simulink model "ACT_ur10"  (R2021b)
(part 6 of 6)

t5571 = -t4d.*(t4257+t4274-t5096+t14.*(t1862+t2375+t330.*(-t496-t547+t615+t623+t755+t8.*t37.*(t100-t364))+t2124.*(t100-t364)));
t5573 = t5572.*t2d;
t5574 = t5572.*t3d;
t5575 = t5572.*t4d;
t5584 = t5583.*t2d;
t5585 = t5583.*t3d;
t5586 = t5583.*t4d;
t5604 = t5601.*t6d;
t5612 = t2665+t2848+t2884+t2931+t3229+t3273+t4524+t4593+t4609;
t5616 = t2188+t2614+t2617+t2986+t3283+t3295+t4605+t4731+t4734;
t5624 = t3661+t3691+t5369+t5376;
t5630 = t3424+t3700+t3759+t5296+t5297;
t5633 = t4477+t4478+t5280+t5288;
t5637 = t2691+t2900+t2902+t4527+t4657+t4660+t5218;
t5641 = t4203+t4230+t4424+t4792+t4813+t4880;
t5642 = t2721+t2899+t2971+t4564+t4684+t4689+t5218;
t5648 = t2814+t3138+t3144+t3608+t3818+t3820+t5101+t5117;
t5652 = t2661+t2842+t2867+t4519+t4614+t4623+t4635+t4649;
t5653 = t2815+t3139+t3143+t3653+t3865+t3914+t5126+t5139;
t5654 = t2970+t3100+t3125+t4209+t4248+t4746+t4795+t4807;
t5662 = t2994+t3076+t3165+t4209+t4248+t4758+t4816+t4839;
t5663 = t2709+t2882+t2901+t4542+t4610+t4619+t4673+t4679;
t5664 = t2887+t3181+t3187+t3673+t3969+t4021+t5135+t5162;
t5665 = -t2d.*(t2845+t3136-t3187-t3673-t3969+t4015-t5135+t5158./2.0);
t5666 = -t3d.*(t2845+t3136-t3187-t3673-t3969+t4015-t5135+t5158./2.0);
t5667 = -t4d.*(t2845+t3136-t3187-t3673-t3969+t4015-t5135+t5158./2.0);
t5669 = t5668.*t1d;
t5671 = t833+t4661+t4662+t4663+t5152+t5231;
t5672 = -t5d.*(t3413+t3663-t3717-t4462-t4463+t4501+t4633./2.0+t4655./2.0);
t5678 = t3009+t3124+t3162+t4406+t4419+t4766+t4852+t4857;
t5681 = t2054+t2427+t2463+t2963+t2982+t3140+t3166+t3337+t3373+t4750+t4817+t4829;
t5688 = t2205+t5240+t5241+t5242+t5272;
t5689 = t2205+t5237+t5238+t5239+t5272;
t5690 = t3670+t3839+t3858+t3960+t3967+t5048+t5132+t5154;
t5693 = -t6d.*(-t2810-t3112+t3146+t3629+t3961-t5142+(t330.*(t1862+t2375+t330.*(-t496-t547+t615+t623+t755+t8.*t37.*(t100-t364))+t2124.*(t100-t364)))./2.0+(t18.*t39.*(t1873+t2355+t2471+t3579))./2.0+(t38.*t39.*(t2068-t2488))./2.0);
t5694 = t6d.*(-t2810-t3112+t3146+t3629+t3961-t5142+(t330.*(t1862+t2375+t330.*(-t496-t547+t615+t623+t755+t8.*t37.*(t100-t364))+t2124.*(t100-t364)))./2.0+(t18.*t39.*(t1873+t2355+t2471+t3579))./2.0+(t38.*t39.*(t2068-t2488))./2.0);
t5695 = t3694+t3926+t3955+t3958+t4006+t5062+t5167+t5183;
t5697 = t3672+t3928+t3975+t4961+t5074+t5186+t5190;
t5700 = -t6d.*(t3735+t3991+t4006./2.0-t4996+t5062./2.0+t5181+t5194);
t5701 = t6d.*(t3735+t3991+t4006./2.0-t4996+t5062./2.0+t5181+t5194);
t5702 = t2850+t3279+t3314+t3736+t3996+t4013+t5082+t5195+t5201;
t5707 = t3552+t3863+t3915+t4729+t4742+t5038+t5105+t5119;
t5708 = t1357+t4987+t4988+t4989+t5338+t5375;
t5712 = t3597+t3900+t3947+t4037+t4278+t4310+t5041+t5110+t5131;
t5713 = t3379+t3632+t3703+t4490+t4633+t4655+t5284+t5294;
t5724 = -t2d.*(t3408-t3662+t3702-t4498+t4675-t5371+t5378+t255.*(t1929-t1996+t2033+t1187.*(t101-t401)));
t5725 = -t3d.*(t3408-t3662+t3702-t4498+t4675-t5371+t5378+t255.*(t1929-t1996+t2033+t1187.*(t101-t401)));
t5726 = -t4d.*(t3408-t3662+t3702-t4498+t4675-t5371+t5378+t255.*(t1929-t1996+t2033+t1187.*(t101-t401)));
t5728 = t3659+t3913+t3917+t5051+t5073+t5086+t5176+t5182;
t5731 = t3420+t5316+t5317+t5318+t5473;
t5732 = -t5d.*(t3398+t5470+t2d.*(t1046+t1185+t1189+t1434-t3519+t158.*t789+t515.*t789+(t8.*(t1609-t2416))./2.0)+t3d.*(t1046+t1185+t1189+t1434-t3519+t158.*t789+t515.*t789+(t8.*(t1609-t2416))./2.0)+t4d.*(t1046+t1185+t1189+t1434-t3519+t158.*t789+t515.*t789+(t8.*(t1609-t2416))./2.0));
t5733 = t5d.*(t3398+t5470+t2d.*(t1046+t1185+t1189+t1434-t3519+t158.*t789+t515.*t789+(t8.*(t1609-t2416))./2.0)+t3d.*(t1046+t1185+t1189+t1434-t3519+t158.*t789+t515.*t789+(t8.*(t1609-t2416))./2.0)+t4d.*(t1046+t1185+t1189+t1434-t3519+t158.*t789+t515.*t789+(t8.*(t1609-t2416))./2.0));
t5741 = -t5d.*(-t2846-t3274-t3277-t3710+t3971+t4036+t4343+t4369+t5156+(t37.*(-t1537+t1983+t3892+t18.*t37.*(t544-t1021+t330.*(t100-t364))))./2.0+(t8.*t37.*(t1070.*(t100-t364)+t330.*(t544-t1021+t330.*(t100-t364))))./2.0+(t14.*t39.*(t1585+t2193-t4001+t38.*t39.*(t544-t1021+t330.*(t100-t364))))./2.0);
t5742 = t5d.*(-t2846-t3274-t3277-t3710+t3971+t4036+t4343+t4369+t5156+(t37.*(-t1537+t1983+t3892+t18.*t37.*(t544-t1021+t330.*(t100-t364))))./2.0+(t8.*t37.*(t1070.*(t100-t364)+t330.*(t544-t1021+t330.*(t100-t364))))./2.0+(t14.*t39.*(t1585+t2193-t4001+t38.*t39.*(t544-t1021+t330.*(t100-t364))))./2.0);
t5765 = t4210+t4240+t4364+t4413+t4446+t5356+t5377+t5382;
t5766 = t4116+t4247+t4291+t4311+t4484+t4489+t5264+t5293+t5299;
t5768 = t4373+t4417+t4429+t4441+t4445+t5355+t5384+t5388;
t2922 = -t2903;
t2924 = -t2905;
t3470 = -t3447;
t4821 = t4808.*t5d;
t4823 = t4809.*t5d;
t4910 = t4904.*t2d;
t4911 = t4904.*t3d;
t4912 = t4904.*t4d;
t4965 = -t4963;
t4999 = t2888+t3255+t3300;
t5205 = t1247+t1648+t1649+t2301+t2689+t2707;
t5232 = t3436+t3772+t3795;
t5274 = t5273.*t5d;
t5332 = t5326.*t2d;
t5333 = t5326.*t3d;
t5334 = t5326.*t4d;
t5339 = t5331.*t2d;
t5340 = t5331.*t3d;
t5341 = t5331.*t4d;
t5347 = -t5344;
t5390 = t5387.*t2d;
t5391 = t5387.*t3d;
t5392 = t5387.*t4d;
t5405 = t5404.*t5d;
t5412 = t5411.*t1d;
t5415 = t2907+t3303+t3333+t4915;
t5417 = -t6d.*(-t2907+t3293+t3324-t3867+t14.*(t1070.*(t100-t364)+t330.*(t544-t1021+t330.*(t100-t364))));
t5420 = t5416.*t5d;
t5421 = t6d.*(-t2907+t3293+t3324-t3867+t14.*(t1070.*(t100-t364)+t330.*(t544-t1021+t330.*(t100-t364))));
t5423 = t5419.*t5d;
t5444 = t5443.*t2d;
t5445 = t5443.*t3d;
t5446 = t5443.*t4d;
t5456 = t301+t4031+t4032+t4033+t4791;
t5472 = -t5469;
t5474 = -t5471;
t5479 = t5477.*t5d;
t5488 = t5487.*t2d;
t5489 = t5487.*t3d;
t5490 = t5487.*t4d;
t5493 = t5492.*t5d;
t5495 = t3448+t3814+t3837+t5243;
t5496 = -t6d.*(-t3448+t3801+t3824-t4411+t14.*(t2578.*(t100-t364)+t609.*(t544-t1021+t330.*(t100-t364))));
t5497 = t6d.*(-t3448+t3801+t3824-t4411+t14.*(t2578.*(t100-t364)+t609.*(t544-t1021+t330.*(t100-t364))));
t5499 = t5498.*t6d;
t5509 = t3438+t3664+t3731+t4594+t4608;
t5510 = t5508.*t5d;
t5518 = t2468+t2668+t2683+t2946+t4184+t4320+t4323;
t5519 = t2466+t2669+t2676+t2947+t4181+t4316+t4318;
t5524 = t2099+t2476+t2506+t3001+t3353+t3396+t5147;
t5527 = t5525.*t6d;
t5530 = t5529.*t2d;
t5531 = t5529.*t3d;
t5532 = t5529.*t4d;
t5535 = t5533.*t2d;
t5536 = t5533.*t3d;
t5537 = t5533.*t4d;
t5538 = t5534.*t2d;
t5539 = t5534.*t3d;
t5540 = t5534.*t4d;
t5541 = t4405+t5455;
t5547 = t2923+t3217+t3239+t3713+t3998+t4035+t4422;
t5553 = t5550.*t5d;
t5563 = t4044+t4305+t4329+t4717+t4725;
t5566 = t5565.*t5d;
t5568 = t4263+t4289+t5096+t5104;
t5587 = t2872+t3190+t3201+t3646+t3842+t3847+t4245+t4262;
t5590 = t2873+t3184+t3205+t3689+t3891+t3946+t4235+t4249;
t5592 = t2079+t2243+t2363+t3294+t3549+t3576+t4814+t4835;
t5599 = t4124+t4344+t4350+t4363+t4421+t4433;
t5606 = t4340+t4496+t4497+t4918+t4919;
t5609 = t2625+t2808+t2830+t3952+t3977+t4515+t4586+t4601;
t5613 = t5612.*t5d;
t5615 = t3990+t4071+t4084+t4694+t4716+t4986;
t5631 = t5630.*t5d;
t5634 = t5633.*t2d;
t5635 = t5633.*t3d;
t5636 = t5633.*t4d;
t5639 = t3446+t3645+t3655+t3714+t3742+t4507+t4686+t4699;
t5643 = t5642.*t6d;
t5649 = t5648.*t2d;
t5650 = t5648.*t3d;
t5651 = t5648.*t4d;
t5655 = t5653.*t2d;
t5656 = t5653.*t3d;
t5657 = t5653.*t4d;
t5658 = t2886+t3180+t3188+t3631+t3911+t3964+t5127+t5134;
t5670 = t3425+t3676+t3717+t4462+t4463+t4502+t4640+t4659;
t5673 = t5671.*t1d;
t5677 = t3017+t3137+t3240+t3411+t3793+t3816+t4772+t4854+t4866;
t5682 = t5681.*t5d;
t5683 = t2080+t2428+t2520+t2968+t3004+t3126+t3192+t3338+t3339+t4767+t4834+t4847;
t5692 = t3644+t3932+t3973+t4962+t5043+t5142+t5171;
t5698 = t5697.*t6d;
t5699 = t3748+t4000+t4012+t4996+t5066+t5185+t5199;
t5703 = t5702.*t6d;
t5704 = t1356+t4972+t4973+t4974+t5329+t5367;
t5709 = t5708.*t1d;
t5715 = t5713.*t2d;
t5716 = t5713.*t3d;
t5717 = t5713.*t4d;
t5723 = t3434+t3662+t3723+t4498+t4677+t4681+t5371+t5380;
t5727 = t3616+t3886+t3945+t5040+t5080+t5089+t5130+t5163;
t5730 = -t5d.*(-t3389+t5469+t2d.*(t1045+t1183+t1184+t1440-t3514+t155.*t788+t508.*t788+(t14.*(t1597-t2409))./2.0)+t3d.*(t1045+t1183+t1184+t1440-t3514+t155.*t788+t508.*t788+(t14.*(t1597-t2409))./2.0)+t4d.*(t1045+t1183+t1184+t1440-t3514+t155.*t788+t508.*t788+(t14.*(t1597-t2409))./2.0));
t5734 = t3386+t3665+t3719+t4123+t4276+t4313+t5266+t5310+t5322;
t5740 = t2846+t3274+t3277+t3710+t3985+t3997+t4043+t4354+t4380+t5057+t5148+t5160;
t5743 = t2847+t3276+t3316+t3711+t3988+t3992+t4053+t4358+t4359+t5075+t5161+t5174;
t5747 = -t2d.*(t3241+t5471+t2d.*(t3350-t3369)+t3d.*(t3350-t3369)+t4d.*(t3350-t3369)+t6d.*(t2098+t2330./2.0+t2351+t3264./2.0-t3507+t3541-t4797));
t5748 = -t3d.*(t3241+t5471+t2d.*(t3350-t3369)+t3d.*(t3350-t3369)+t4d.*(t3350-t3369)+t6d.*(t2098+t2330./2.0+t2351+t3264./2.0-t3507+t3541-t4797));
t5749 = -t4d.*(t3241+t5471+t2d.*(t3350-t3369)+t3d.*(t3350-t3369)+t4d.*(t3350-t3369)+t6d.*(t2098+t2330./2.0+t2351+t3264./2.0-t3507+t3541-t4797));
t5750 = t2d.*(t3241+t5471+t2d.*(t3350-t3369)+t3d.*(t3350-t3369)+t4d.*(t3350-t3369)+t6d.*(t2098+t2330./2.0+t2351+t3264./2.0-t3507+t3541-t4797));
t5751 = t3d.*(t3241+t5471+t2d.*(t3350-t3369)+t3d.*(t3350-t3369)+t4d.*(t3350-t3369)+t6d.*(t2098+t2330./2.0+t2351+t3264./2.0-t3507+t3541-t4797));
t5752 = t4d.*(t3241+t5471+t2d.*(t3350-t3369)+t3d.*(t3350-t3369)+t4d.*(t3350-t3369)+t6d.*(t2098+t2330./2.0+t2351+t3264./2.0-t3507+t3541-t4797));
t5758 = t4106+t4223+t4260+t4927+t4928+t5261+t5287+t5295;
t5767 = t5766.*t5d;
t5769 = t3437+t3823+t3825+t4384+t4444+t4465+t5359+t5386+t5393;
t5771 = t1792+t5300+t5301+t5302+t5431+t5448;
t5774 = t5399+t5731;
t5775 = -t5d.*(t3398-t5399+t5470+t2d.*(t1046+t1185+t1189+t1434-t3519+t158.*t789+t515.*t789+(t8.*(t1609-t2416))./2.0)+t3d.*(t1046+t1185+t1189+t1434-t3519+t158.*t789+t515.*t789+(t8.*(t1609-t2416))./2.0)+t4d.*(t1046+t1185+t1189+t1434-t3519+t158.*t789+t515.*t789+(t8.*(t1609-t2416))./2.0));
t5776 = t5d.*(t3398-t5399+t5470+t2d.*(t1046+t1185+t1189+t1434-t3519+t158.*t789+t515.*t789+(t8.*(t1609-t2416))./2.0)+t3d.*(t1046+t1185+t1189+t1434-t3519+t158.*t789+t515.*t789+(t8.*(t1609-t2416))./2.0)+t4d.*(t1046+t1185+t1189+t1434-t3519+t158.*t789+t515.*t789+(t8.*(t1609-t2416))./2.0));
t5785 = t3435+t3773+t3836+t4328+t4382+t4430+t4455+t4511+t4516+t5357+t5379+t5383;
t5003 = t4999.*t6dd;
t5208 = t5205.*t6d;
t5233 = t5232.*t6dd;
t5275 = -t5274;
t5394 = -t5390;
t5395 = -t5391;
t5396 = -t5392;
t5407 = -t5405;
t5414 = -t5412;
t5424 = -t5420;
t5425 = -t5423;
t5457 = t5456.*t1d;
t5500 = -t5499;
t5512 = -t5510;
t5520 = t5518.*t5d;
t5521 = t5519.*t5d;
t5526 = t5524.*t6d;
t5544 = t2922+t3223+t3233+t3660+t3957+t3995+t4423;
t5548 = t5547.*t6d;
t5554 = -t5553;
t5564 = t5563.*t5d;
t5567 = -t5566;
t5588 = t5587.*t5d;
t5591 = t5590.*t5d;
t5594 = t5592.*t2d;
t5595 = t5592.*t3d;
t5596 = t5592.*t4d;
t5598 = t2924+t3315+t3317+t4051+t4365+t4383+t4895;
t5602 = t5599.*t6d;
t5607 = t5606.*t5d;
t5614 = -t5613;
t5632 = -t5631;
t5640 = t5639.*t6d;
t5644 = t3470+t3794+t3855+t4191+t4214+t4347+t4518+t4523;
t5646 = t1083+t4821+t5191+t5192+t5193;
t5647 = t1084+t4823+t5196+t5197+t5198;
t5659 = t5658.*t2d;
t5660 = t5658.*t3d;
t5661 = t5658.*t4d;
t5674 = t3010+t3182+t3204+t4756+t4849+t4851+t5232;
t5679 = t5677.*t6d;
t5684 = t5683.*t5d;
t5705 = t5704.*t1d;
t5710 = -t5709;
t5729 = t3389+t5319+t5320+t5321+t5472;
t5735 = t5734.*t6d;
t5736 = t2874+t5007+t5008+t5009+t5277+t5493;
t5744 = t5743.*t5d;
t5746 = t3257+t4637+t4638+t4639+t5474+t5504;
t5753 = t3296+t4690+t4691+t4692+t5479+t5507;
t5755 = -t2d.*(t3270-t5479-t5507+t2d.*(t3442+(t14.*(t1864-t2028))./2.0)+t3d.*(t3442+(t14.*(t1864-t2028))./2.0)+t4d.*(t3442+(t14.*(t1864-t2028))./2.0));
t5756 = -t3d.*(t3270-t5479-t5507+t2d.*(t3442+(t14.*(t1864-t2028))./2.0)+t3d.*(t3442+(t14.*(t1864-t2028))./2.0)+t4d.*(t3442+(t14.*(t1864-t2028))./2.0));
t5757 = -t4d.*(t3270-t5479-t5507+t2d.*(t3442+(t14.*(t1864-t2028))./2.0)+t3d.*(t3442+(t14.*(t1864-t2028))./2.0)+t4d.*(t3442+(t14.*(t1864-t2028))./2.0));
t5770 = t5769.*t6d;
t5772 = t5771.*t1d;
t5786 = t5785.*t5d;
t5792 = t3393+t5484+t5485+t5486+t5497+t5511;
t5794 = t4630+t5535+t5536+t5537+t5618;
t5797 = t1031+t2500+t2502+t2504+t3378+t5246+t5247+t5248+t5349+t5730;
t5798 = t1081+t2499+t2501+t2503+t3358+t5252+t5253+t5254+t5347+t5733;
t5799 = t2890+t5422+t5530+t5531+t5532+t5552;
t5811 = -t5d.*(t4520+t5613+t2d.*(-t2021+t2249+t3374+t3395+t4569-t4577+t37.*(t1580+t2001)+t8.*t37.*t1503.*(t100-t364))+t3d.*(-t2021+t2249+t3374+t3395+t4569-t4577+t37.*(t1580+t2001)+t8.*t37.*t1503.*(t100-t364))+t4d.*(-t2021+t2249+t3374+t3395+t4569-t4577+t37.*(t1580+t2001)+t8.*t37.*t1503.*(t100-t364))+t6d.*(t2675+t2885-t3385+t3633-t3680-t4527+t4656-t4657+(t892.*t2198)./2.0));
t5812 = t4543+t5560+t5561+t5562+t5622+t5643;
t5823 = t5044+t5649+t5650+t5651+t5694+t5718;
t5825 = t5070+t5655+t5656+t5657+t5698+t5721;
t5236 = -t5233;
t5522 = -t5520;
t5528 = -t5526;
t5545 = t5544.*t6d;
t5549 = -t5548;
t5576 = t2203+t3775+t3776+t3777+t5407;
t5589 = -t5588;
t5593 = -t5591;
t5600 = t5598.*t6d;
t5605 = -t5602;
t5608 = -t5607;
t5645 = t5644.*t6d;
t5676 = t5674.*t6d;
t5680 = -t5679;
t5706 = -t5705;
t5722 = t5208+t5689;
t5737 = -t5735;
t5738 = t5736.*t6d;
t5745 = -t5744;
t5754 = t2129+t5275+t5440+t5441+t5442;
t5759 = t4219+t5332+t5333+t5334+t5521;
t5791 = t2984+t5425+t5450+t5451+t5452+t5527;
t5793 = t3393+t5488+t5489+t5490+t5497+t5512;
t5795 = t5794.*t5d;
t5800 = t2834+t5421+t5538+t5539+t5540+t5554;
t5801 = t4510+t5335+t5336+t5337+t5640+t5672;
t5809 = t4079+t5567+t5573+t5574+t5575+t5604;
t5810 = t4525+t5556+t5557+t5558+t5614+t5638;
t5813 = t5812.*t5d;
t5815 = t3327+t5500+t5625+t5626+t5627+t5632;
t5824 = t5823.*t5d;
t5826 = t5825.*t5d;
t5827 = t5071+t5659+t5660+t5661+t5701+t5742;
t5830 = -t6d.*(t5088-t5703+t5744+t2d.*(t2845+t3136-t3187-t3673-t3969+t4015-t5135+t5158./2.0)+t3d.*(t2845+t3136-t3187-t3673-t3969+t4015-t5135+t5158./2.0)+t4d.*(t2845+t3136-t3187-t3673-t3969+t4015-t5135+t5158./2.0));
t5835 = t5363+t5724+t5725+t5726+t5770+t5786;
t5546 = -t5545;
t5577 = t5576.*t2d;
t5578 = t5576.*t3d;
t5579 = t5576.*t4d;
t5603 = -t5600;
t5739 = -t5738;
t5760 = t4211+t5339+t5340+t5341+t5522;
t5761 = t5759.*t5d;
t5781 = t3692+t4910+t4911+t4912+t5549+t5593;
t5790 = t2939+t5424+t5444+t5445+t5446+t5528;
t5796 = -t5795;
t5802 = t5801.*t2d;
t5803 = t5801.*t3d;
t5804 = t5801.*t4d;
t5814 = -t5813;
t5816 = t4753+t5584+t5585+t5586+t5676+t5682;
t5819 = t4761+t5594+t5595+t5596+t5680+t5684;
t5821 = t4368+t5608+t5634+t5635+t5636+t5645;
t5828 = t5827.*t6d;
t5829 = t5095+t5665+t5666+t5667+t5703+t5745;
t5832 = t5271+t5715+t5716+t5717+t5737+t5767;
t5836 = t5835.*t6d;
t5580 = -t5577;
t5581 = -t5578;
t5582 = -t5579;
t5762 = t5760.*t5d;
t5763 = -t5761;
t5777 = t3657+t4884+t4885+t4886+t5546+t5589;
t5782 = t5781.*t2d;
t5783 = t5781.*t3d;
t5784 = t5781.*t4d;
t5805 = -t5802;
t5806 = -t5803;
t5807 = -t5804;
t5808 = t4062+t5564+t5569+t5570+t5571+t5603;
t5817 = t5816.*t6d;
t5820 = t5819.*t6d;
t5822 = t1081+t2499+t2501+t2503+t3236+t3358+t5394+t5395+t5396+t5414+t5739+t5776;
t5833 = t5832.*t5d;
t5837 = -t5836;
t5764 = -t5762;
t5778 = t5777.*t2d;
t5779 = t5777.*t3d;
t5780 = t5777.*t4d;
t5788 = t982+t2997+t3725+t3727+t3729+t5324+t5763;
t5818 = -t5817;
t5831 = t2130+t4009+t4010+t4011+t4557+t5457+t5580+t5581+t5582+t5796;
t5834 = -t5833;
t5839 = t2026+t3635+t3637+t3639+t4399+t4479+t5673+t5755+t5756+t5757+t5814+t5820;
t5841 = t2759+t4447+t4448+t4449+t4966+t5004+t5710+t5782+t5783+t5784+t5826+t5830;
t5789 = t983+t2998+t3726+t3728+t3730+t5323+t5764;
t5838 = t1940+t3636+t3638+t3640+t4400+t4480+t5669+t5750+t5751+t5752+t5811+t5818;
t5840 = t2758+t4434+t4436+t4438+t4965+t5003+t5706+t5778+t5779+t5780+t5824+t5828;
t5842 = t3361+t4818+t4819+t4820+t5220+t5236+t5772+t5805+t5806+t5807+t5834+t5837;
et1 = -t2d.*(t4d.*(t2467+t2490+t3177+t3185)-t3d.*(t2956+t2989+t3349+t3351)-t2d.*(-t8.*t1302.*t2174+t14.*t1302.*t2168+t8.*t1321.*t2659+t14.*t1321.*t2655)+t5d.*(t2070+t2085-t2937-t2951))+t1d.*(-t5d.*(t706.*t2655.*2.0+t723.*t2659.*2.0)+t4d.*(t1288.*t2655.*2.0-t1298.*t2659.*2.0)+t3d.*(t1962.*t2655.*2.0-t1977.*t2659.*2.0)+t2d.*(t2168.*t2655.*2.0-t2174.*t2659.*2.0))+t4491.*t4dd+t4596.*t3dd+t4695.*t2dd-t5018.*t5dd-t4d.*(t3d.*(t2606+t2642+t3177+t3185)+t2d.*(t2745+t2775+t3177+t3185)+t4d.*(t3177+t3185-t14.*t687.*t1288+t8.*t687.*t1298)+t5d.*(t1547+t1574-t2937-t2951));
et2 = -t3d.*(t4d.*(t2286+t2346+t3177+t3185)-t2d.*(t2995+t3007+t3349+t3351)-t3d.*(t3349+t3351+t14.*t1036.*t1962-t8.*t1036.*t1977)+t5d.*(t1837+t1866-t2937-t2951))+t1dd.*(t2655.^2+t2659.^2)+t5d.*(t2d.*(t3840+t3875+t4579+t4591)+t4d.*(t3331+t4579+t4591+t1288.*(t859-t1704))+t3d.*(t3712+t4579+t4591+t1962.*(t859-t1704))+t5d.*(t723.*t2507+t1399.*t2655-t706.*(t859-t1704)-t2659.*(t441-t846)));
et3 = -t2d.*(t4d.*(t3183+t3214+t3781+t3785)+t3d.*(t3557+t3574+t3972+t3976)-t2d.*(-t8.*t2173.*t2279+t14.*t2167.*t2279+t8.*t2357.*t2658+t14.*t2357.*t2654)+t5d.*(t2862+t2876-t3359-t3360))-t6dd.*(t2658.*(t873-t2434)+t2654.*(t910-t2473))+t1d.*(-t5d.*(t705.*t2654.*2.0+t721.*t2658.*2.0)+t4d.*(t1287.*t2654.*2.0-t1297.*t2658.*2.0)+t3d.*(t1961.*t2654.*2.0-t1976.*t2658.*2.0)+t2d.*(t2167.*t2654.*2.0-t2173.*t2658.*2.0))+t4878.*t4dd+t4946.*t3dd+t4967.*t2dd-t5219.*t5dd-t5787.*t6d+t5d.*(t2d.*(t4166+t4189+t4931+t4938)+t5d.*(t721.*t3230+t705.*t3251+t2123.*t2654+t2169.*t2658)+t4d.*(t3923-t3936+t4931+t4938)+t3d.*(t4125-t4128+t4931+t4938));
et4 = -t4d.*(t3d.*(t3308+t3321+t3781+t3785)+t2d.*(t3415+t3445+t3781+t3785)+t4d.*(t3781+t3785-t14.*t1287.*t1807+t8.*t1297.*t1807)+t5d.*(t2509+t2527-t3359-t3360))-t3d.*(t4d.*(t3035+t3069+t3781+t3785)+t2d.*(t3575+t3617+t3972+t3976)+t3d.*(t3972+t3976-t14.*t1961.*t2113+t8.*t1976.*t2113)+t5d.*(t2708+t2718-t3359-t3360))+t1dd.*(t2654.^2+t2658.^2);
et5 = -t5dd.*(t37.*t418+t14.*t496.*t641+t8.*t496.*(t100-t364))-t6dd.*(t18.*t552-t641.*t698+t733.*(t100-t364))+t418.*t1dd+t2213.*t2dd+t2213.*t3dd+t2213.*t4dd-t5432.*t2d-t5432.*t3d-t5432.*t4d-t1d.*(-t861+t341.*t403.*t2d.*2.0+t341.*t403.*t3d.*2.0+t341.*t403.*t4d.*2.0+t18.*t61.*t341.*t5d.*2.0);
et6 = -t5d.*(t4174+t2d.*(-t552-t961+t1264+t2180+t8.*t494.*(t100-t364)+t14.*t39.*(t844-t1156))+t3d.*(-t552-t961+t1264+t2180+t8.*t494.*(t100-t364)+t14.*t39.*(t844-t1156))+t4d.*(-t552-t961+t1264+t2180+t8.*t494.*(t100-t364)+t14.*t39.*(t844-t1156))-t5d.*(t232.*t341.*2.0-t14.*t39.*t1738+t8.*t39.*t1780))-t6d.*(t4337-t5d.*(t187.*t341.*2.0-t12.*t552-t641.*t732+t255.*t1738+t330.*t1780+t699.*(t100-t364))+t4846.*t2d+t4846.*t3d+t4846.*t4d);
et7 = -t1d.*(t861+t342.*t402.*t2d.*2.0+t342.*t402.*t3d.*2.0+t342.*t402.*t4d.*2.0-t18.*t63.*t402.*t5d.*2.0)-t5dd.*(t37.*t446+t8.*t548.*t609+t14.*t548.*(t101-t401))-t6d.*(-t4337+t5d.*(t12.*t598+t215.*t402+t609.*t763+t255.*t1786+t330.*t1742+t759.*(t101-t401))+t2d.*(t632-t1007+t1328-t2402+t627.*(t101-t401)+t330.*(t952-t1028))+t3d.*(t632-t1007+t1328-t2402+t627.*(t101-t401)+t330.*(t952-t1028))+t4d.*(t632-t1007+t1328-t2402+t627.*(t101-t401)+t330.*(t952-t1028)))-t6dd.*(t18.*t598+t609.*t760-t735.*(t101-t401))+t446.*t1dd-t2292.*t2dd;
et8 = -t2292.*t3dd-t2292.*t4dd+t5435.*t2d+t5435.*t3d+t5435.*t4d-t5d.*(-t4174+t2d.*(-t598-t962+t1284+t2235+t14.*t546.*(t101-t401)+t8.*t39.*(t952-t1028))+t3d.*(-t598-t962+t1284+t2235+t14.*t546.*(t101-t401)+t8.*t39.*(t952-t1028))+t4d.*(-t598-t962+t1284+t2235+t14.*t546.*(t101-t401)+t8.*t39.*(t952-t1028))+t5d.*(t233.*t402.*2.0+t8.*t39.*t1742-t14.*t39.*t1786));
et9 = -t3762.*t2dd-t3762.*t3dd-t3762.*t4dd-t4164.*t5dd-t4324.*t6dd-t5d.*(t5d.*(t37.*(t602-t639)-t14.*t39.*(t729-t785-t806+t18.*t61.*(t101-t401))+t8.*t39.*(t752-t781-t838+t18.*t63.*(t100-t364)))+t2d.*(-t964-t1903+t2339+t3521+t3558+t14.*t37.*(t1155+t341.*(t101-t401)))+t3d.*(-t964-t1903+t2339+t3521+t3558+t14.*t37.*(t1155+t341.*(t101-t401)))+t4d.*(-t964-t1903+t2339+t3521+t3558+t14.*t37.*(t1155+t341.*(t101-t401)))-t6d.*(t37.*t1044-t8.*t39.*t2190+t14.*t39.*t2259));
et10 = -t2d.*(t3788+t2d.*(t3478-t3506)+t3d.*(t3478-t3506)+t4d.*(t3478-t3506)+t5d.*(t8.*(t729-t785-t806+t18.*t61.*(t101-t401))+t14.*(t752-t781-t838+t18.*t63.*(t100-t364))))-t3d.*(t3788+t2d.*(t3478-t3506)+t3d.*(t3478-t3506)+t4d.*(t3478-t3506)+t5d.*(t8.*(t729-t785-t806+t18.*t61.*(t101-t401))+t14.*(t752-t781-t838+t18.*t63.*(t100-t364))));
et11 = -t4d.*(t3788+t2d.*(t3478-t3506)+t3d.*(t3478-t3506)+t4d.*(t3478-t3506)+t5d.*(t8.*(t729-t785-t806+t18.*t61.*(t101-t401))+t14.*(t752-t781-t838+t18.*t63.*(t100-t364))))-t1d.*(t1044.*t6d+t1776.*t2d+t1776.*t3d+t1776.*t4d-t5d.*(t602-t639));
et12 = -t6d.*(t5361.*t2d+t5361.*t3d+t5361.*t4d+t5d.*(t329.*(t1155+t341.*(t101-t401))+t255.*(t729-t785-t806+t18.*t61.*(t101-t401))+t330.*(t752-t781-t838+t18.*t63.*(t100-t364))+t402.*t543.*2.0-t256.*t2189+t18.*t39.*(t602-t639))+t6d.*(t255.*t2259+t330.*t2190-t18.*t39.*t1044))+t341.*t402.*t1dd.*2.0;
et13 = t6d.*(t2d.*(t696+t1464-t1849+t1905-t2940+t330.*(t582+t616-t761+t18.*t37.*(t100-t364)))+t3d.*(t696+t1464-t1849+t1905-t2940+t330.*(t582+t616-t761+t18.*t37.*(t100-t364)))+t4d.*(t696+t1464-t1849+t1905-t2940+t330.*(t582+t616-t761+t18.*t37.*(t100-t364)))+t3826.*t6d-t5d.*(t200.*t341+t256.*t1699+t329.*t1663+t255.*t2171+t330.*t2170+t18.*t39.*t930))+t5d.*(t3620.*t6d+t5125.*t2d+t5125.*t3d+t5125.*t4d-t5d.*(t37.*t930+t8.*t39.*t2170-t14.*t39.*t2171))-t544.*t1dd.*2.0+t3057.*t2dd+t3057.*t3dd+t3057.*t4dd+t3595.*t5dd+t3808.*t6dd-t5481.*t2d-t5481.*t3d-t5481.*t4d;
et14 = -t1d.*(t591.*t6d.*2.0-t930.*t5d+t1289.*t2d+t1289.*t3d+t1289.*t4d);
et15 = t1d.*(t544.*t6d.*2.0-t949.*t5d+t2d.*(t569-t604)+t3d.*(t569-t604)+t4d.*(t569-t604))-t591.*t1dd.*2.0+t3058.*t2dd+t3058.*t3dd+t3058.*t4dd+t3620.*t5dd+t3826.*t6dd+t5491.*t2d+t5491.*t3d+t5491.*t4d-t5d.*(t2d.*(t645-t1815+t1832-t2857-t2891+t37.*(t569-t604))+t3d.*(t645-t1815+t1832-t2857-t2891+t37.*(t569-t604))+t4d.*(t645-t1815+t1832-t2857-t2891+t37.*(t569-t604))-t5d.*(t37.*t949+t8.*t39.*t2204+t14.*t39.*(-t537+t759+t12.*t39.*(t101-t401)))+t3595.*t6d);
et16 = t6d.*(-t3808.*t6d+t2d.*(t711.*2.0+t1465+t1844+t1960+t3011+t3029)+t3d.*(t711.*2.0+t1465+t1844+t1960+t3011+t3029)+t4d.*(t711.*2.0+t1465+t1844+t1960+t3011+t3029)-t5d.*(t200.*t402+t256.*t1659+t329.*t1701-t330.*t2204+t255.*(-t537+t759+t12.*t39.*(t101-t401))-t18.*t39.*t949));
et17 = t244+t404-t2719.*t1dd+t4301.*t3dd+t3d.*(t2406+t2d.*(t896+t897+t900+t932+t3271+t3326)+t3d.*(-t2610-t2961+t69.*t530.*5.723e-1+t71.*t530.*5.723e-1+t2361.*(t890+t8.*(t553-t8.*t15.*(1.53e+2./2.5e+2)))))+t2dd.*(t23.*t562+t26.*t562+t1935.^2)-t1d.*(t2407+t2796.*t2d+t1d.*((t299.*t928)./1.0e+4-t553.*t793));
et18 = t2d.*(t3d.*(-t897-t932-t2610.*2.0+t3258+t69.*t530.*8.5845e-1+t71.*t530.*8.5845e-1+(t1935.*(t890+t8.*(t553-t8.*t15.*(1.53e+2./2.5e+2))))./2.0)+t2796.*t1d+t2d.*(-t1265.*t1935+t23.*t529.*t530+t26.*t529.*t530));
et19 = t244+t404+t420-t2d.*(t4950.*t1d+t3d.*(t1751+t1755+t4170-t2300.*t3083.*(3.0./2.0)+t23.*t670.*t820.*(3.0./2.0)+t26.*t670.*t820.*(3.0./2.0))+t4d.*(t1375+t1378-t3580.*2.0+t4539+t4540+t108.*t820.*1.22925e-1+t113.*t820.*1.22925e-1)-t2d.*(t2666.*t3083+t23.*t820.*t843+t26.*t820.*t843))+t4025.*t1dd+t4917.*t3dd+t5001.*t4dd-t1d.*(-t4950.*t2d+t3d.*(t2044+t2074-t2122+t2136+t2393+t2395)+t1d.*(t1410.*t1674-t1413.*t1677)+t4d.*(t1733-t1741+t3432))+t2dd.*(t23.*t880+t26.*t880+t3083.^2);
et20 = -t4d.*(t3d.*(t1123+t1134+t1135+t1139+t1331+t1334+t4394+t4460+t4464)+t4d.*(t1331+t1334+t3613+t4095+t3383.*t3750)-t2d.*(t1355+t1358+t1375+t1378+t4539+t4540)-t1d.*(-t1733+t1741+t3432))+t3d.*(t1d.*(t2122-t2136+t2393+t2395)+t2d.*(t1751-t1754+t1755-t1758+t4170+t4176)-t4d.*(t1094+t1098+t1172+t1174+t1331+t1334+t3335+t3613+t4459+t4460)-t3d.*(-t2300.*t3083+t23.*t670.*t820+t26.*t670.*t820));
et21 = t244+t404+t419+t443+t493+t4695.*t1dd+t5343.*t3dd+t5360.*t4dd+t5dd.*(-t3348+t4873+t14.*t1302.*(t859-t1704))-t2d.*(-t5d.*(t3384+t3399+t4325+t4327+t4546.*2.0+t4665+t5178+t12.*t108.*t1302.*1.157e-1+t12.*t113.*t1302.*1.157e-1)+t5292.*t1d+t3d.*(t2398+t2400+t4930+t3405.*t4155.*(3.0./2.0)-t23.*t1055.*t1302.*(3.0./2.0)-t26.*t1055.*t1302.*(3.0./2.0))+t4d.*(t2100.*(3.0./2.0)+t2101.*(3.0./2.0)+t2141+t2142+t4741.*2.0+t5069+t5084)-t2d.*(-t3687.*t4155+t23.*t1302.*t1321+t26.*t1302.*t1321))+t2dd.*(t23.*t1333+t26.*t1333+t4155.^2);
et22 = -t1d.*(-t5292.*t2d+t4d.*(t2467+t2490-t2780+t2790+t3231+t3237)-t3d.*(t2956+t2989+t3014-t3018+t3380+t3381)+t1d.*(t2168.*t2655-t2174.*t2659)+t5d.*(t2070+t2085+t2953+t2966+t3872+t3903+t4595+t4604));
et23 = t5d.*(-t1d.*(t3872+t3903+t4595+t4604)+t2d.*(-t3384+t4321+t4332-t4665+t5173+(t14.*t1321.*(t859-t1704))./2.0)+t3d.*(-t3298+t4236+t4237+t4299-t4553+t5098+t5165+t14.*t1302.*(t855-t885-t1427+t1706)+(t14.*t1055.*(t859-t1704))./2.0)+t4d.*(t3079+t3087+t4151+t4152+t4267+t4299+t4861+t5165+t5228+t14.*t1302.*(t855-t885-t1427+t1706))-t5d.*(t4027+t4547+t4551+t4923+t1875.*t4155+t34.*t39.*t2507.*5.785e-2-t14.*t1302.*t1399+t8.*t1302.*(t441-t846)-t36.*t39.*(t859-t1704).*5.785e-2));
et24 = t3d.*(-t1d.*(-t3014+t3018+t3380+t3381)+t5d.*(t1517+t1520+t1709+t1713+t3298+t3306+t4236+t4237+t4451+t4546+t4553+t5098)-t4d.*(t1965+t1968+t1969+t1973+t2100+t2101+t4642+t4741+t5026+t5028)+t2d.*(t2398+t2399+t2400+t2401+t4930+t4936)+t3d.*(-t3405.*t4155+t23.*t1055.*t1302+t26.*t1055.*t1302))+t4d.*(-t4d.*(t2100+t2101+t4741+t4900+t4131.*t4428)+t1d.*(t2780-t2790+t3231+t3237)+t3d.*(t1965+t1968+t1969+t1973-t2100-t2101+t4991-t5026+t5028)+t5d.*(t1245+t1248+t1709+t1713+t3090+t3101+t4151+t4152+t4546+t4770+t4861+t5228)+t2d.*(t2141+t2142+t2155+t2156+t5069+t5084));
et25 = t244+t404+t419+t442+t492+t4967.*t1dd+t5408.*t3dd+t5433.*t4dd-t5434.*t5dd-t6dd.*(t4674+t8.*t2279.*(t873-t2434)+t14.*t2279.*(t910-t2473))+t2dd.*(t23.*t2311+t26.*t2311+t4154.^2);
et26 = t6d.*(t5465+t4d.*(t3943-t4666+t4694+t4716-t4776-t4798-t4879+t4986+(t8.*t1818.*(t873-t2434))./2.0+(t14.*t1818.*(t910-t2473))./2.0)+t5523.*t1d-t5641.*t2d+t3d.*(t4367+t4757+t4765-t4776-t4798+t4833-t4879+(t8.*t2140.*(t873-t2434))./2.0+(t14.*t2140.*(t910-t2473))./2.0)-t5d.*(-t4707-t4971+t5686+t2270.*(t745-t747)+t8.*t2279.*(t870-t909-t1470+t2472)+t8.*t1082.*(t873-t2434)+t14.*t1082.*(t910-t2473)));
et27 = -t5d.*(t5687+t1d.*(t4186+t4201+t4941+t4947)-t3d.*(t4188+t4192-t4552+t4874+t4875+t4881+t4888+t5097+t5164)+t5d.*(t3843+t3848+t4026+t4922+t5011+t5012+t1874.*t4154-t14.*t2123.*t2279-t8.*t2169.*t2279)-t4d.*(t4118+t4121+t4266+t4840+t4841+t4860+t4881+t4888+t5164+t5227)+t2d.*(t4290+t4296+t4664+t4890+t4891+t5177))-t1d.*(-t5403.*t2d-t5523.*t6d+t4d.*(t3183+t3214-t3456+t3469+t3809+t3812)+t3d.*(t3557+t3574-t3622+t3630+t4002+t4003)+t5d.*(t2862+t2876-t3359-t3360+t4186+t4201+t4941+t4947)+t1d.*(t2167.*t2654-t2173.*t2658));
et28 = -t4d.*(t2d.*(t3543+t3544-t3578-t3582-t5068+t5077)+t3d.*(t3452+t3457+t3458+t3459+t3516+t3517+t4983+t5025+t5029)+t4d.*(t3516+t3517+t4740+t4899+t4130.*t4427)-t1d.*(t3456-t3469+t3809+t3812)-t5d.*(t2743+t2744+t3086+t3088+t4122+t4127+t4545+t4769+t4840+t4841+t4860+t5227)+t6d.*(t4666+t4700+t4721+t4982+(t8.*t1818.*(t873-t2434))./2.0+(t14.*t1818.*(t910-t2473))./2.0));
et29 = -t3d.*(t2d.*(t3745+t3747-t3770-t3771-t4929+t4933)-t1d.*(t3622-t3630+t4002+t4003)-t5d.*(t2983+t2985+t3086+t3088+t4193+t4200+t4450+t4545+t4552+t4874+t4875+t5097)+t4d.*(t3439+t3440+t3472+t3473+t3516+t3517+t4641+t4740+t5025+t5027)+t6d.*(t4367+t4760+t4768+t4830+(t8.*t2140.*(t873-t2434))./2.0+(t14.*t2140.*(t910-t2473))./2.0)+t3d.*(t3404.*t4154+t23.*t2140.*t2279+t26.*t2140.*t2279));
et30 = -t2d.*(t5403.*t1d-t5641.*t6d+t3d.*(t3770+t3771+t4929+t3404.*t4154.*(3.0./2.0)+t23.*t2140.*t2279.*(3.0./2.0)+t26.*t2140.*t2279.*(3.0./2.0))-t5d.*(t3086.*2.0+t3088.*2.0+t4290+t4296+t4545.*2.0+t4664+t4890+t4891+t5177)+t4d.*(t3516.*(3.0./2.0)+t3517.*(3.0./2.0)+t3578+t3582+t4740.*2.0+t5068+t5083)-t2d.*(-t3686.*t4154+t23.*t2279.*t2357+t26.*t2279.*t2357));
et31 = t404+t2d.*(t2406+t2d.*(t2610+t346.*t529+t347.*t529-t1265.*t2361-t1935.*(t890+t8.*(t553-t8.*t15.*(1.53e+2./2.5e+2))))+t3d.*(t896+t900-t2645-t3000+t31.*t69.*1.63763645e-1+t31.*t71.*1.63763645e-1))-t2374.*t1dd+t4301.*t2dd;
et32 = t3d.*(t2406+t2d.*(-t896-t900+t2645+t3000+t31.*t69.*4.91290935e-1+t31.*t71.*4.91290935e-1-t2361.*(t890+t8.*(t553-t8.*t15.*(1.53e+2./2.5e+2))).*2.0)+t3d.*(-t2961+t31.*t69.*3.2752729e-1+t31.*t71.*3.2752729e-1))+t3dd.*(t23.*t42.*3.2752729e-1+t26.*t42.*3.2752729e-1+t2361.^2)-t1d.*(t2407+t2372.*t2d-t1d.*(t308.*t793+t315.*t824));
et33 = t404+t420+t3d.*(t4785.*t1d+t2d.*(t1754+t1758+t4185+t2300.*t2749.*(3.0./2.0)-t23.*t647.*t670.*(3.0./2.0)-t26.*t647.*t670.*(3.0./2.0))-t4d.*(t1172+t1174-t3318.*2.0+t4256+t4459+t108.*t647.*1.22925e-1+t113.*t647.*1.22925e-1)-t3d.*(-t2300.*t2749+t23.*t647.*t670+t26.*t647.*t670))+t3817.*t1dd+t4917.*t2dd+t4920.*t4dd-t1d.*(t4785.*t3d+t2d.*(t2075+t2090-t2093+t2119+t2393+t2395)+t1d.*(t1121.*t1674-t1140.*t1677)+t4d.*(t1499-t1501+t3432));
et34 = -t2d.*(t3d.*(t1754+t1758+t4185-(t2300.*t2749)./2.0+(t23.*t647.*t670)./2.0+(t26.*t647.*t670)./2.0)-t1d.*(-t2090+t2093+t2393+t2395)+t4d.*(t1093+t1097+t1172+t1174+t1332+t1335+t3335+t3613+t4395+t4459)-t2d.*(t2666.*t2749+t23.*t647.*t843+t26.*t647.*t843))+t3dd.*(t23.*t675+t26.*t675+t2749.^2)-t4d.*(t2d.*(t1093+t1097+t1123+t1134+t1355+t1358+t4395+t4457+t4464)+t3d.*(t1094+t1098+t1123+t1134-t4256+t4464)+t4d.*(t1093+t1097+t3335+t4095+t2813.*t3750)-t1d.*(-t1499+t1501+t3432));
et35 = t404+t419+t443+t493-t5d.*(t1d.*(t3751+t4595+t4604+(t1962.*(t859-t1704))./2.0)+t4d.*(t3090+t3101+t4149+t4212+t4221+t4252-t4714+t5093-t5228+(t14.*t687.*(t855-t885-t1427+t1706))./2.0)+t2d.*(t3298+t3306+t4212+t4221+t4321+t4332+t4553+t5093+t5173)-t5d.*(t4538-t4551-t4923+t1875.*t4050+t3082.*(t746-t748)+t14.*t1036.*t1399-t34.*t39.*t2507.*5.785e-2-t8.*t1036.*(t441-t846)+t39.*t219.*(t859-t1704))+t3d.*(t3298+t3306+t4236+t4237+t4553+t5098))+t4596.*t1dd+t5343.*t2dd+t5345.*t4dd-t5351.*t5dd;
et36 = t4d.*(t2d.*(-t1889-t1891+t1965+t1969+t2144+t2145+t4995+t5020+t5028)-t4d.*(t1889+t1891+t4642+t4900+t3822.*t4428)+t1d.*(t2644-t2648+t3231+t3237)+t5d.*(t1245+t1248+t1517+t1520+t3090+t3101+t4151+t4152+t4451+t4714+t4770+t5228)+t3d.*(t1965+t1969+t1995+t1999+t4957+t5028))+t2d.*(-t4d.*(t1889+t1891+t1965+t1969+t2144+t2145+t4642+t4741-t4995+t5028)+t3d.*(t2399+t2401+t4936+(t3405.*t4050)./2.0+(t23.*t1036.*t1055)./2.0+(t26.*t1036.*t1055)./2.0)-t1d.*(t2996-t2999+t3380+t3381)+t5d.*(t1517+t1520+t1709+t1713+t3298+t3306+t4325+t4327+t4451+t4546+t4553+t5178)+t2d.*(t3687.*t4050+t23.*t1036.*t1321+t26.*t1036.*t1321))+t3dd.*(t23.*t1096+t26.*t1096+t4050.^2);
et37 = -t1d.*(-t5255.*t3d+t4d.*(t2286+t2346-t2644+t2648+t3231+t3237)-t2d.*(t2995-t2996+t2999+t3007+t3380+t3381)+t1d.*(t1962.*t2655-t1977.*t2659)+t5d.*(t1837+t1866+t2953+t2966+t3751+t4595+t4604+(t1962.*(t859-t1704))./2.0))+t3d.*(t2d.*(-t2399-t2401+t4934+t3405.*t4050.*(3.0./2.0)+t23.*t1036.*t1055.*(3.0./2.0)+t26.*t1036.*t1055.*(3.0./2.0))-t5255.*t1d-t4d.*(t1889.*(3.0./2.0)+t1891.*(3.0./2.0)+t1965+t1969-t4627.*2.0+t4957+t5028)+t5d.*(t3298+t3306+t4236+t4237+t4553+t5098-t4050.*(t746-t748).*2.0+t12.*t108.*t1036.*1.157e-1+t12.*t113.*t1036.*1.157e-1)+t3d.*(t3405.*t4050+t23.*t1036.*t1055+t26.*t1036.*t1055));
et38 = t404+t419+t442+t492-t1d.*(t5397.*t3d-t5515.*t6d+t4d.*(t3035+t3069+t3330-t3332+t3809+t3812)+t2d.*(t3575+t3598-t3601+t3617+t4002+t4003)+t1d.*(t1961.*t2654-t1976.*t2658)+t5d.*(t2708+t2718-t3359-t3360+t4136-t4137+t4941+t4947));
et39 = t6d.*(t5465+t5515.*t1d-t5d.*(-t4668+t4935+t5686+t2270.*(t745-t747)+t8.*t2113.*(t870-t909-t1470+t2472)+t8.*t1082.*(t873-t2434)+t14.*t1082.*(t910-t2473))+t4d.*(t3943-t4487+t4694+t4716-t4747-t4759+t4815+t4986+(t8.*t1818.*(t873-t2434))./2.0+(t14.*t1818.*(t910-t2473))./2.0)+t3d.*(t4367+t4760+t4768+t4830+(t8.*t2140.*(t873-t2434))./2.0+(t14.*t2140.*(t910-t2473))./2.0)+t2d.*(t4367-t4747-t4759+t4792+t4813+t4815+t4880+(t8.*t2140.*(t873-t2434))./2.0+(t14.*t2140.*(t910-t2473))./2.0))+t4946.*t1dd+t5408.*t2dd+t5410.*t4dd-t5413.*t5dd;
et40 = t5d.*(t3d.*(t4188+t4192-t4552+t4870-t4875-t5097)+t5d.*(-t3843-t3848-t4922+t5006-t5011+t1874.*t4049+t3081.*(t745-t747)+t14.*t2113.*t2123+t8.*t2113.*t2169)-t2d.*(t4193+t4200+t4552+t4865+t4867+t4889+t4892+t5092+t5172)-t1d.*(t4136-t4137+t4941+t4947)+t4d.*(t4118+t4121+t4266+t4713+t4840+t4841+t4862-t4865-t5092+t5227)+t6d.*(t4476+t4784+t4954+t4960+t4992+t5000));
et41 = t2d.*(-t4d.*(t3400+t3401+t3472+t3473+t3543+t3544+t4641+t4740-t4994+t5027)-t3d.*(t3745+t3747+t4933-(t3404.*t4049)./2.0+(t23.*t2113.*t2140)./2.0+(t26.*t2113.*t2140)./2.0)+t1d.*(-t3598+t3601+t4002+t4003)+t5d.*(t2983+t2985+t3086+t3088+t4193+t4200+t4450+t4545+t4552+t4890+t4891+t5177)+t6d.*(t4146+t4157+t4371+t4792+t4813+t4880)+t2d.*(t3686.*t4049+t23.*t2113.*t2357+t26.*t2113.*t2357))+t3dd.*(t23.*t2147+t26.*t2147+t4049.^2);
et42 = t4d.*(t2d.*(-t3400-t3401+t3472+t3473+t3543+t3544+t4994+t5019+t5027)-t3d.*(t3439+t3440+t3452+t3458-t4956+t5029)-t4d.*(t3400+t3401+t4641+t4899+t3821.*t4427)+t1d.*(-t3330+t3332+t3809+t3812)+t5d.*(t2743+t2744+t2983+t2985+t4122+t4127+t4450+t4713+t4769+t4840+t4841+t5227)-t6d.*(t4487+t4700+t4721+t4982+(t8.*t1818.*(t873-t2434))./2.0+(t14.*t1818.*(t910-t2473))./2.0));
et43 = t3d.*(t5629+t5d.*(t2983.*2.0+t2985.*2.0+t4193+t4200+t4552+t4874+t4875+t5097-t4049.*(t745-t747).*2.0)+t5397.*t1d+t2d.*(t3745+t3747+t4933+t3404.*t4049.*(3.0./2.0)-t23.*t2113.*t2140.*(3.0./2.0)-t26.*t2113.*t2140.*(3.0./2.0))-t4d.*(t3400.*(3.0./2.0)+t3401.*(3.0./2.0)+t3472+t3473-t4626.*2.0+t4956+t5027)-t3d.*(-t3404.*t4049+t23.*t2113.*t2140+t26.*t2113.*t2140))-t6dd.*(-t4561+t8.*t2113.*(t873-t2434)+t14.*t2113.*(t910-t2473));
et44 = t420+t3429.*t1dd+t4920.*t3dd+t5001.*t2dd-t1d.*(t3432.*t4d+t3d.*(t1500+t1516+t3432)+t2d.*(t1740+t1759+t3432)+t1d.*(t37.*t1736.*8.195e-2-t325.*t1677))+t2d.*(t3461-t4d.*(t648+t652+t1332+t1335-t3623+t4108)-t3d.*(t1122+t1133+t1135+t1139+t1332+t1335+t3340+t3623+t4394+t4454)+t2d.*(t3613+t392.*t843+t393.*t843+t2666.*t3750+t3083.*t3383))-t4d.*(t3483+t3d.*(t649+t653+t1135+t1139+t3340+t4101-t2813.*t3750.*2.0)+t2d.*(t649+t653+t1355+t1358+t3623+t4101-t3383.*t3750.*2.0)+t4d.*(t4095+t39.*t104.*6.7158025e-3+t39.*t107.*6.7158025e-3));
et45 = t4dd.*(t23.*t53.*6.7158025e-3+t26.*t53.*6.7158025e-3+t3750.^2)-t3d.*(t3483+t4d.*(t648+t652+t1094+t1098-t3340+t4108)+t3d.*(t1122+t1133+t3318+t4454-t2749.*t2813)+t2d.*(t1094+t1098+t1122+t1133+t1355+t1358+t3340+t3623+t4454+t4457));
et46 = t419+t443+t493+t3d.*(t3d.*(t1888+t1890+t4642+t5022+t3822.*t4050)+t1d.*(t2348-t2359+t3231+t3237)+t5d.*(t1245+t1248+t1517+t1520+t3090+t3101+t4236+t4237+t4283+t4451+t4770+t5098)+t2d.*(t1888+t1890+t1995+t1999+t2144+t2145+t4652+t4752+t5020+t5022)-t4d.*(t1650+t1652+t1968+t1973+t4652+t4906))-t4d.*(t4d.*(t4900+t23.*t687.*t703+t26.*t687.*t703)+t3d.*(t1651+t1653+t1995+t1999+t4647+t4902-t3822.*t4428.*2.0)-t5081.*t1d+t2d.*(t1651+t1653+t2155+t2156-t4752+t4902-t4131.*t4428.*2.0)-t5d.*(t3090+t3101+t4151+t4152+t4283+t5228-t4428.*(t746-t748).*2.0+t12.*t108.*t687.*1.157e-1+t12.*t113.*t687.*1.157e-1))+t4491.*t1dd+t5345.*t3dd+t5360.*t2dd-t5366.*t5dd;
et47 = t2d.*(t1d.*(-t2508+t2511+t3231+t3237)+t5d.*(t1245+t1248+t1709+t1713+t3090+t3101+t4283+t4325+t4327+t4546+t4770+t5178)+t2d.*(t4741+t3687.*t4428-t4131.*t4155+t23.*t687.*t1321+t26.*t687.*t1321)+t3d.*(t1888+t1890+t1968+t1973+t2155+t2156+t4652+t4752+t4991+t5022)-t4d.*(t1650+t1652+t2144+t2145+t4752+t4906))+t4dd.*(t23.*t720+t26.*t720+t4428.^2)-t1d.*(t5081.*t4d+t3d.*(-t2348+t2359+t2606+t2642+t3231+t3237)+t2d.*(t2508-t2511+t2745+t2775+t3231+t3237)+t1d.*(t1288.*t2655-t1298.*t2659)+t5d.*(t1547+t1574+t2953+t2966+t3355+t4595+t4604+(t1288.*(t859-t1704))./2.0));
et48 = -t5d.*(t1d.*(t3355+t4595+t4604+(t1288.*(t859-t1704))./2.0)+t2d.*(t3090+t3101+t4139+t4143-t4283+t4321+t4332+t4856+t5173+t5226)+t3d.*(t3090+t3101+t4139+t4143+t4231-t4283+t4704-t5098+t5226+(t14.*t1036.*(t855-t885-t1427+t1706))./2.0)-t5d.*(t4538-t4551-t4923+t1875.*t4428+t3082.*(t746-t748)+t14.*t687.*t1399-t34.*t39.*t2507.*5.785e-2-t8.*t687.*(t441-t846)+t36.*t39.*(t859-t1704).*5.785e-2)+t4d.*(t3090+t3101+t4151+t4152+t4283+t5228));
et49 = t419+t442+t492-t1d.*(t5327.*t4d-t5505.*t6d+t3d.*(-t3073+t3080+t3308+t3321+t3809+t3812)+t2d.*(t3232-t3234+t3415+t3445+t3809+t3812)+t1d.*(t1287.*t2654-t1297.*t2658)+t5d.*(t2509+t2527-t3359-t3360+t3965-t3978+t4941+t4947));
et50 = t6d.*(t5465+t5505.*t1d+t3d.*(t3990+t4475-t4678-t4705+t4757+t4765+t4833+t4977+(t8.*t1818.*(t873-t2434))./2.0+(t14.*t1818.*(t910-t2473))./2.0)+t2d.*(t3990+t4648-t4678-t4705+t4792+t4813+t4880+t4977+(t8.*t1818.*(t873-t2434))./2.0+(t14.*t1818.*(t910-t2473))./2.0)-t5d.*(-t4582+t5076+t5686+t2270.*(t745-t747)+t8.*t1807.*(t870-t909-t1470+t2472)+t8.*t1082.*(t873-t2434)+t14.*t1082.*(t910-t2473))+t4d.*(t3982+t4700+t4721+t4982+(t8.*t1818.*(t873-t2434))./2.0+(t14.*t1818.*(t910-t2473))./2.0))+t4878.*t1dd+t5410.*t3dd+t5433.*t2dd-t5437.*t5dd;
et51 = t5d.*(t4d.*(t4118+t4121-t4282+t4838-t4841-t5227)+t5d.*(-t3843-t3848-t4922+t5006-t5011+t1874.*t4427+t3081.*(t745-t747)+t14.*t1807.*t2123+t8.*t1807.*t2169)-t1d.*(t3965-t3978+t4941+t4947)+t3d.*(t4118+t4121+t4282-t4703+t4831-t4836+t4874+t4875+t5097-t5225)+t2d.*(t4118+t4121+t4282+t4831-t4836-t4855+t4890+t4891+t5177-t5225)+t6d.*(t4476+t4784+t4954+t4960+t4992+t5000));
et52 = -t3d.*(t2d.*(t3414+t3416+t3439+t3440-t3543-t3544+t4646-t4751-t5019+t5024)+t3d.*(t3414+t3416+t4626+t5024-t3821.*t4049)-t1d.*(t3073-t3080+t3809+t3812)-t5d.*(t2743+t2744+t2983+t2985+t4122+t4127+t4282+t4450+t4769+t4874+t4875+t5097)+t6d.*(t3982+t4760+t4768+t4830+(t8.*t1818.*(t873-t2434))./2.0+(t14.*t1818.*(t910-t2473))./2.0)+t4d.*(t3288+t3291+t3439+t3440+t4651+t4905))+t4dd.*(t23.*t1840+t26.*t1840+t4427.^2);
et53 = t4d.*(t5d.*(t2743.*2.0+t2744.*2.0+t4122+t4127+t4282+t4840+t4841+t5227-t4427.*(t745-t747).*2.0)-t4d.*(t4899+t23.*t1807.*t1818+t26.*t1807.*t1818)-t3d.*(t3289+t3292+t3457+t3459+t4646+t4901-t3821.*t4427.*2.0)+t5327.*t1d-t6d.*(t3982+t4700+t4721+t4982+(t8.*t1818.*(t873-t2434))./2.0+(t14.*t1818.*(t910-t2473))./2.0)+t2d.*(-t3289-t3292+t3543+t3544+t4751+t4905+t4130.*t4427.*2.0))-t6dd.*(-t4868+t8.*t1807.*(t873-t2434)+t14.*t1807.*(t910-t2473));
et54 = -t2d.*(t3d.*(t3414+t3416+t3457+t3459+t3543+t3544+t4646-t4751+t4983+t5024)-t1d.*(-t3232+t3234+t3809+t3812)-t5d.*(t2743+t2744+t3086+t3088+t4122+t4127+t4282+t4545+t4769+t4890+t4891+t5177)-t2d.*(t4740+t3686.*t4427-t4130.*t4154+t23.*t1807.*t2357+t26.*t1807.*t2357)+t4d.*(t3288+t3291+t3543+t3544+t4751+t4905)+t6d.*(t3982-t4792-t4813-t4880+(t8.*t1818.*(t873-t2434))./2.0+(t14.*t1818.*(t910-t2473))./2.0));
et55 = t12.*t39.*(-5.675085e-1)-t5018.*t1dd-t5351.*t3dd-t5366.*t4dd+t2dd.*(-t3348+t4873+t14.*t1302.*(t859-t1704))-t2d.*(-t1d.*(t2117+t2128+t2954+t2967)-t5d.*(t2593+t2619+t2781+t2798+t4048-t4572)+t4d.*(t1222+t1246+t1710+t1714+t3066+t3078+t4252+t4304+t4309+t4559+t4783+t5169)+t3d.*(t1518+t1521+t1710+t1714+t3260+t3272+t4304+t4309+t4468+t4534+t4559+t5169)+t2d.*(t1709+t1713+t4304+t4309+t4546+t5169+t3082.*t3687+t8.*t1321.*t2507-t14.*t1321.*(t859-t1704)));
et56 = -t4d.*(-t1d.*(t1618+t1636+t2954+t2967)+t4d.*(t1245+t1248+t3066+t3078+t4139+t4143+t4252+t4770+t5226)+t3d.*(t1222+t1246+t1518+t1521+t3066+t3078+t4139+t4143+t4468+t4704+t4783+t5226)+t2d.*(t1222+t1246+t1710+t1714+t3066+t3078+t4139+t4143+t4559+t4783+t4856+t5226)-t5d.*(t2178+t2206+t2781+t2798+t4048+t4825))-t3d.*(-t1d.*(t1930+t1944+t2954+t2967)+t3d.*(t1517+t1520+t3260+t3272+t4212+t4221+t4451+t4534+t5093)+t4d.*(t1222+t1246+t1518+t1521+t3066+t3078+t4212+t4221+t4252+t4468+t4783+t5093)+t2d.*(t1518+t1521+t1710+t1714+t3260+t3272+t4212+t4221+t4468+t4534+t4559+t5093)-t5d.*(t2438+t2478+t2781+t2798+t4048+t4494));
et57 = -t5d.*(t4d.*(t2178+t2206+t2781+t2798+t4048+t4541-t4556+t4825-t4926)-t2d.*(t2608+t2630+t2772+t2779+t4042+t4548+t4556+t4572+t4926)+t5283.*t1d-t5d.*(-t1875.*t3082+t2507.*(t441-t846)+t1399.*(t859-t1704))+t3d.*(t2438+t2781+t2798+t4048+t4494+t4541-t4556-t4926-(t8.*t1036.*(t441-t846))./2.0))+t1d.*(t5283.*t5d+t1d.*(t706.*t2655+t723.*t2659)+t2d.*(t2117+t2128+t2954+t2967+t3840+t3875+t4579+t4591)+t4d.*(t1618+t1636+t2954+t2967+t3331+t4579+t4591+t1288.*(t859-t1704))+t3d.*(t1930+t1944+t2954+t2967+t3712+t4579+t4591+t1962.*(t859-t1704)))+t5dd.*((t859-t1704).^2+t2507.^2+t3082.^2);
et58 = -t5482.*t1d+t5619.*t5d+t4d.*(-t4599+t5090+t5685+(t2270.*(t745-t747))./2.0+(t8.*t1807.*(t870-t909-t1470+t2472))./2.0+(t8.*t1082.*(t873-t2434))./2.0+(t14.*t1082.*(t910-t2473))./2.0)+t3d.*(-t4672+t4943+t5685+(t2270.*(t745-t747))./2.0+(t8.*t2113.*(t870-t909-t1470+t2472))./2.0+(t8.*t1082.*(t873-t2434))./2.0+(t14.*t1082.*(t910-t2473))./2.0)+t2d.*(-t4720-t4976+t5685+(t2270.*(t745-t747))./2.0+(t8.*t2279.*(t870-t909-t1470+t2472))./2.0+(t8.*t1082.*(t873-t2434))./2.0+(t14.*t1082.*(t910-t2473))./2.0);
et59 = t6d.*(t2270.*t3734+t4178.*(t910-t2473)-(t873-t2434).*(t870-t909-t1470+t2472));
et60 = -t5d.*(t3d.*(t3590+t3628+t3894+t3901+t4047+t4493-t4925+t5010-t5014)+t4d.*(t3421+t3468+t3894+t3901+t4047+t4824-t4925+t5010-t5014)+t5d.*(t1874.*t3081+t2123.*t3251+t2169.*t3230)-t2d.*(t3716+t3756+t3874+t3890+t4041+t4571+t4925+t5013+t5014)+t5401.*t1d+t5619.*t6d)-t12.*t39.*1.356723-t5219.*t1dd-t5413.*t3dd-t5434.*t2dd-t5437.*t4dd;
et61 = t4d.*(t6d.*(-t4599+t5090+(t2270.*(t745-t747))./2.0+(t8.*t1807.*(t870-t909-t1470+t2472))./2.0+(t8.*t1082.*(t873-t2434))./2.0+(t14.*t1082.*(t910-t2473))./2.0)-t4d.*(t2743+t2744+t4115+t4117+t4251+t4769+t4836+t4837+t5225)-t3d.*(t2776+t2777+t3012+t3013+t4115+t4117+t4467+t4703+t4782+t4836+t4837+t5225)-t2d.*(t2776+t2777+t3129+t3130+t4115+t4117+t4558+t4782+t4836+t4837+t4855+t5225)+t1d.*(t2557+t2576-t3387-t3390)+t5d.*(t3421+t3468+t3894+t3901+t4047+t4824));
et62 = t3d.*(t6d.*(-t4672+t4943+(t2270.*(t745-t747))./2.0+(t8.*t2113.*(t870-t909-t1470+t2472))./2.0+(t8.*t1082.*(t873-t2434))./2.0+(t14.*t1082.*(t910-t2473))./2.0)-t3d.*(t2983+t2985+t4183+t4187+t4450+t4533+t4865+t4867+t5092)-t4d.*(t2776+t2777+t3012+t3013+t4115+t4117+t4251+t4467+t4782+t4865+t4867+t5092)-t2d.*(t3012+t3013+t3129+t3130+t4183+t4187+t4467+t4533+t4558+t4865+t4867+t5092)+t1d.*(t2747+t2755-t3387-t3390)+t5d.*(t3590+t3628+t3894+t3901+t4047+t4493))+t6d.*(et58+et59);
et63 = t2d.*(t5d.*(t3701+t3741+t3894+t3901+t4047-t4571)+t6d.*(-t4720-t4976+(t2270.*(t745-t747))./2.0+(t8.*t2279.*(t870-t909-t1470+t2472))./2.0+(t8.*t1082.*(t873-t2434))./2.0+(t14.*t1082.*(t910-t2473))./2.0)-t4d.*(t2776+t2777+t3129+t3130+t4115+t4117+t4251+t4558+t4782+t4883+t4887+t5168)-t3d.*(t3012+t3013+t3129+t3130+t4183+t4187+t4467+t4533+t4558+t4883+t4887+t5168)-t2d.*(t3086+t3088+t4545+t4883+t4887+t5168+t3081.*t3686+t8.*t2357.*t3230+t14.*t2357.*t3251)+t1d.*(t2915+t2929-t3387-t3390))+t5dd.*(t3081.^2+t3230.^2+t3251.^2);
et64 = t1d.*(t5401.*t5d-t5482.*t6d+t2d.*(t2915+t2929-t3387-t3390+t4166+t4189+t4931+t4938)+t1d.*(t705.*t2654+t721.*t2658)+t4d.*(t2557+t2576-t3387-t3390+t3923-t3936+t4931+t4938)+t3d.*(t2747+t2755-t3387-t3390+t4125-t4128+t4931+t4938))+t6dd.*(-t4156+t3230.*(t873-t2434)+t3251.*(t910-t2473));
et65 = t6d.*(t4093+t4224+t4253+(t330.*(t2574+t1532.*(t100-t364)))./2.0-(t543.*t2198)./2.0+(t1066.*t2198)./2.0-(t1068.*t2198)./2.0-(t255.*t3862)./2.0+(t18.*t39.*t3591)./2.0)+t2d.*(-t2625+t2797-t3952-t4515+t4576+t4588+(t14.*(t2574+t1532.*(t100-t364)))./2.0+t8.*t37.*t2198.*(t100-t364))+t3d.*(-t2625+t2797-t3952-t4515+t4576+t4588+(t14.*(t2574+t1532.*(t100-t364)))./2.0+t8.*t37.*t2198.*(t100-t364))+t4d.*(-t2625+t2797-t3952-t4515+t4576+t4588+(t14.*(t2574+t1532.*(t100-t364)))./2.0+t8.*t37.*t2198.*(t100-t364));
et66 = -t5d.*((t37.*t3591)./2.0+(t8.*t39.*(t2574+t1532.*(t100-t364)))./2.0+(t14.*t39.*t3862)./2.0)-t1d.*(t1916./2.0+t2376./2.0);
et67 = t2d.*(t2647+t2829-t4519-t4614+t4634-t4635+(t14.*(t3377.*(t100-t364)+t13.*t330.*(t544-t1021+t330.*(t100-t364))))./2.0+t892.*t2198)+t3d.*(t2647+t2829-t4519-t4614+t4634-t4635+(t14.*(t3377.*(t100-t364)+t13.*t330.*(t544-t1021+t330.*(t100-t364))))./2.0+t892.*t2198)+t4d.*(t2647+t2829-t4519-t4614+t4634-t4635+(t14.*(t3377.*(t100-t364)+t13.*t330.*(t544-t1021+t330.*(t100-t364))))./2.0+t892.*t2198);
et68 = t6d.*(t4105+t4319+t4345+(t330.*(t3377.*(t100-t364)+t13.*t330.*(t544-t1021+t330.*(t100-t364))))./2.0-(t255.*t4575)./2.0-(t543.*(t544-t1021+t330.*(t100-t364)))./2.0+(t1066.*(t544-t1021+t330.*(t100-t364)))./2.0-(t1068.*(t544-t1021+t330.*(t100-t364)))./2.0+(t18.*t39.*t4506)./2.0)+t5d.*(-t330.*(t2574+t1532.*(t100-t364))+t543.*t2198+t1016.*t2198+t1068.*t2198+t255.*t3862+(t37.*t4506)./2.0+(t8.*t39.*(t3377.*(t100-t364)+t13.*t330.*(t544-t1021+t330.*(t100-t364))))./2.0-t18.*t39.*t3591+(t14.*t39.*t4575)./2.0);
et69 = -t1d.*(t2724./2.0+t3604./2.0);
et70 = t5d.*(et65+et66)+t5dd.*(t494.*t2198+t764.*t2198+t802.*t2198)+t6dd.*(t544.*t2198-t1021.*t2198+t2526.*(t100-t364))-t4182.*t2dd-t4182.*t3dd-t4182.*t4dd-t5790.*t2d-t5790.*t3d-t5790.*t4d+t6d.*(et67+et68+et69);
et71 = -t1d.*(t2d.*(t1838+t1892-t2583+t341.*(-t496-t547+t615+t623+t755+t8.*t37.*(t100-t364)))+t3d.*(t1838+t1892-t2583+t341.*(-t496-t547+t615+t623+t755+t8.*t37.*(t100-t364)))+t4d.*(t1838+t1892-t2583+t341.*(-t496-t547+t615+t623+t755+t8.*t37.*(t100-t364)))-t5d.*(t3591-t232.*t341+(t14.*t39.*t1738)./2.0-(t8.*t39.*t1780)./2.0)+t6d.*(t4068+t187.*t341-(t12.*t552)./2.0-(t641.*t732)./2.0+(t255.*t1738)./2.0+(t330.*t1780)./2.0+(t699.*(t100-t364))./2.0)-t18.*t61.*t341.*t1d)-t341.*t2198.*t1dd;
et72 = t5dd.*(t546.*t2233+t726.*t2233+t871.*t2233)+t6dd.*(t591.*t2233+t1015.*t2233+t1069.*t2233);
et73 = t6d.*(t2d.*(t2690+t2841-t4542-t4610-t4619+t4670-t4673+t937.*t2233)+t3d.*(t2690+t2841-t4542-t4610-t4619+t4670-t4673+t937.*t2233)+t4d.*(t2690+t2841-t4542-t4610-t4619+t4670-t4673+t937.*t2233)-t6d.*(t4105+t4319+t4345+(t588.*t2578)./2.0-(t969.*t2578)./2.0+(t1193.*t2578)./2.0+(t255.*t4587)./2.0+(t330.*t4578)./2.0+(t18.*t39.*t4508)./2.0)+t1d.*(t2703./2.0+t3625./2.0)+t5d.*(t255.*(t2550-t1535.*(t101-t401))+t588.*t2233-t969.*t2233-t1137.*t2233+t330.*t3866-(t37.*t4508)./2.0+t18.*t39.*t3634-(t8.*t39.*t4578)./2.0+(t14.*t39.*t4587)./2.0));
et74 = t1d.*(t5030.*t2d+t5030.*t3d+t5030.*t4d-t5d.*(t3634-t233.*t402-(t8.*t39.*t1742)./2.0+(t14.*t39.*t1786)./2.0)+t6d.*(t4068+t191.*t402+t12.*t646-(t609.*t736)./2.0+(t255.*t1786)./2.0+(t330.*t1742)./2.0+(t759.*(t101-t401))./2.0)-t18.*t63.*t402.*t1d)+t4204.*t2dd+t4204.*t3dd+t4204.*t4dd-t5791.*t2d-t5791.*t3d-t5791.*t4d;
et75 = -t5d.*(t2d.*(t2664-t2807+t3953+t3979+t4531+t4631+t4645-t14.*t37.*t2233.*(t101-t401))+t3d.*(t2664-t2807+t3953+t3979+t4531+t4631+t4645-t14.*t37.*t2233.*(t101-t401))+t4d.*(t2664-t2807+t3953+t3979+t4531+t4631+t4645-t14.*t37.*t2233.*(t101-t401))+t6d.*(t4093+t4224+t4253+(t255.*(t2550-t1535.*(t101-t401)))./2.0+(t588.*t2233)./2.0-(t969.*t2233)./2.0+(t1193.*t2233)./2.0+(t330.*t3866)./2.0+(t18.*t39.*t3634)./2.0)-t5d.*((t37.*t3634)./2.0-(t14.*t39.*(t2550-t1535.*(t101-t401)))./2.0+(t8.*t39.*t3866)./2.0)-t1d.*(t1971./2.0+t2414./2.0))-t402.*t2233.*t1dd;
et76 = t1617+t3195+t3196+t3197+t4087+t6dd.*(t137.*t1420+t317.*t1420+t368.*t1420)-t1d.*(t162+t4272+t6d.*(t12.*t138.*(-3.0./2.0)+(t330.*t478)./2.0-(t255.*t1126)./2.0+(t330.*(t478-t519))./2.0+(t18.*t329.*t437)./2.0)+t2d.*(-t1281+t3322+(t14.*(t478-t519))./2.0)+t3d.*(-t1281+t3322+(t14.*(t478-t519))./2.0)+t4d.*(-t1281+t3322+(t14.*(t478-t519))./2.0))+t5722.*t2d+t5722.*t3d+t5722.*t4d;
et77 = t6d.*(t5475.*t2d+t5475.*t3d+t5475.*t4d-t5d.*(t255.*t1784+t330.*t1743+t18.*t2958-t255.*t3104+(t37.*(t1268-t1988))./2.0+t330.*(t1743-t1783)+t18.*t155.*t1420-(t8.*t39.*t3176)./2.0+(t14.*t39.*t3175)./2.0)+t1d.*(t1268./2.0-t1988./2.0)+t6d.*((t255.*t1497)./2.0+(t330.*t1468)./2.0+(t255.*t3175)./2.0+(t330.*t3176)./2.0-(t18.*t112.*t1070)./2.0-(t18.*t39.*(t1268-t1988))./2.0));
et78 = t5d.*(t2962+t5016+t2d.*(-t1586-t1867+t1920-t3218+t3370+t3535+(t14.*(t1743-t1783))./2.0+t14.*t39.*(t1609-t2416))+t3d.*(-t1586-t1867+t1920-t3218+t3370+t3535+(t14.*(t1743-t1783))./2.0+t14.*t39.*(t1609-t2416))+t4d.*(-t1586-t1867+t1920-t3218+t3370+t3535+(t14.*(t1743-t1783))./2.0+t14.*t39.*(t1609-t2416))+t6d.*((t255.*t1784)./2.0+(t330.*t1743)./2.0-t18.*t2973-(t255.*t3104)./2.0+(t330.*(t1743-t1783))./2.0-(t18.*t112.*t1420)./2.0));
et79 = -t1d.*(t2699./2.0-t3607./2.0+t3624./2.0-(t18.*t63.*(t544-t1021+t330.*(t100-t364)))./2.0)+t5773.*t2d+t5773.*t3d+t5773.*t4d+t6d.*(t12.*t4364.*(-1.0./2.0)+t255.*t4196+t330.*t4168-(t329.*t4404)./2.0+(t256.*(t2578.*(t100-t364)+t609.*(t544-t1021+t330.*(t100-t364))))./2.0+(t255.*(t2816+t3757+t3780-t19.*t255.*(t544-t1021+t330.*(t100-t364))))./2.0+(t330.*(t2853+t3739+t3755-t19.*t330.*(t544-t1021+t330.*(t100-t364))))./2.0-t18.*t39.*t4078+(t18.*t39.*t5257)./2.0);
et80 = t5d.*(t12.*t4094-t256.*t4167+t329.*t4195-t255.*t4914-t330.*t4913+(t37.*t5257)./2.0+t18.*t39.*(t1925-t1963+t2378-t2412)-(t14.*t39.*(t2816+t3757+t3780-t19.*t255.*(t544-t1021+t330.*(t100-t364))))./2.0+(t8.*t39.*(t2853+t3739+t3755-t19.*t330.*(t544-t1021+t330.*(t100-t364))))./2.0);
et81 = -t4068.*t1dd+t5147.*t2dd+t5147.*t3dd+t5147.*t4dd+t5821.*t2d+t5821.*t3d+t5821.*t4d+t6d.*(et79+et80)+t5d.*(t5758.*t2d+t5758.*t3d+t5758.*t4d+t5d.*((t37.*(t1925-t1963+t2378-t2412))./2.0-(t8.*t39.*t4913)./2.0+(t14.*t39.*t4914)./2.0)+t1d.*(t1925./2.0-t1963./2.0+t2378./2.0-t2412./2.0)-t6d.*(t37.*t4078+t12.*t4111-(t256.*t4167)./2.0+(t329.*t4195)./2.0-(t255.*t4914)./2.0-(t330.*t4913)./2.0+(t18.*t39.*(t1925-t1963+t2378-t2412))./2.0-t8.*t39.*t4168+t14.*t39.*t4196))+t5dd.*(t4093+t4224+t4253)+t6dd.*(t4105+t4319+t4345);
et82 = t1d.*(t5438.*t2d+t5438.*t3d+t5438.*t4d+t5d.*(t4822+(t37.*(t602-t639))./2.0-(t14.*t39.*(t729-t785-t806+t18.*t61.*(t101-t401)))./2.0+(t8.*t39.*(t752-t781-t838+t18.*t63.*(t100-t364)))./2.0)-t1d.*(t18.*t63.*t341-t18.*t61.*t402)+t6d.*(t4078+(t329.*(t1155+t341.*(t101-t401)))./2.0+(t255.*(t729-t785-t806+t18.*t61.*(t101-t401)))./2.0+(t330.*(t752-t781-t838+t18.*t63.*(t100-t364)))./2.0+t402.*t543-(t256.*t2189)./2.0+(t18.*t39.*(t602-t639))./2.0));
et83 = t6d.*(t3609+t3861+t3919-(t12.*t3552)./2.0+(t256.*t3800)./2.0+(t255.*t4708)./2.0+(t330.*t4715)./2.0-(t329.*(t2068-t2488))./2.0+(t18.*t39.*(t1606+t1678-t1797-t2356))./2.0)-t5d.*((t37.*(t1606+t1678-t1797-t2356))./2.0-(t14.*t39.*t4708)./2.0+(t8.*t39.*t4715)./2.0)-t1d.*(t1606./2.0+t1678./2.0-t1797./2.0-t2356./2.0)+t2d.*(-t3552+t3882+t4726+t4736+t5102+t37.*(t1873+t2355+t2471+t3579)+t8.*t39.*(t1862+t2375+t330.*(-t496-t547+t615+t623+t755+t8.*t37.*(t100-t364))+t2124.*(t100-t364))+t14.*t37.*(t2068-t2488));
et84 = t3d.*(-t3552+t3882+t4726+t4736+t5102+t37.*(t1873+t2355+t2471+t3579)+t8.*t39.*(t1862+t2375+t330.*(-t496-t547+t615+t623+t755+t8.*t37.*(t100-t364))+t2124.*(t100-t364))+t14.*t37.*(t2068-t2488))+t4d.*(-t3552+t3882+t4726+t4736+t5102+t37.*(t1873+t2355+t2471+t3579)+t8.*t39.*(t1862+t2375+t330.*(-t496-t547+t615+t623+t755+t8.*t37.*(t100-t364))+t2124.*(t100-t364))+t14.*t37.*(t2068-t2488));
et85 = t6d.*(t3647+t4005+t4007-(t12.*t3670)./2.0-(t329.*t3833)./2.0+(t255.*t5045)./2.0+(t330.*t5049)./2.0+(t256.*(t1070.*(t100-t364)+t330.*(t544-t1021+t330.*(t100-t364))))./2.0+(t18.*t39.*t4975)./2.0)-t1d.*(t1311./2.0+t2184./2.0+t3475./2.0-(t12.*t39.*(t544-t1021+t330.*(t100-t364)))./2.0)-t5d.*(-t12.*t3552+t256.*t3800+t255.*t4708-(t37.*t4975)./2.0+t330.*t4715-t329.*(t2068-t2488)+t18.*t39.*(t1606+t1678-t1797-t2356)-(t8.*t39.*t5049)./2.0+(t14.*t39.*t5045)./2.0);
et86 = t2d.*(t3592+t3912+t5072+t5085-t5130+t330.*(t1862+t2375+t330.*(-t496-t547+t615+t623+t755+t8.*t37.*(t100-t364))+t2124.*(t100-t364))+t18.*t39.*(t1873+t2355+t2471+t3579)+t38.*t39.*(t2068-t2488))+t3d.*(t3592+t3912+t5072+t5085-t5130+t330.*(t1862+t2375+t330.*(-t496-t547+t615+t623+t755+t8.*t37.*(t100-t364))+t2124.*(t100-t364))+t18.*t39.*(t1873+t2355+t2471+t3579)+t38.*t39.*(t2068-t2488))+t4d.*(t3592+t3912+t5072+t5085-t5130+t330.*(t1862+t2375+t330.*(-t496-t547+t615+t623+t755+t8.*t37.*(t100-t364))+t2124.*(t100-t364))+t18.*t39.*(t1873+t2355+t2471+t3579)+t38.*t39.*(t2068-t2488));
et87 = -t2d.*(-t4062-t5564+t5600+t2d.*(t4257+t4274-t5096+t14.*(t1862+t2375+t330.*(-t496-t547+t615+t623+t755+t8.*t37.*(t100-t364))+t2124.*(t100-t364)))+t3d.*(t4257+t4274-t5096+t14.*(t1862+t2375+t330.*(-t496-t547+t615+t623+t755+t8.*t37.*(t100-t364))+t2124.*(t100-t364)))+t4d.*(t4257+t4274-t5096+t14.*(t1862+t2375+t330.*(-t496-t547+t615+t623+t755+t8.*t37.*(t100-t364))+t2124.*(t100-t364))));
et88 = -t3d.*(-t4062-t5564+t5600+t2d.*(t4257+t4274-t5096+t14.*(t1862+t2375+t330.*(-t496-t547+t615+t623+t755+t8.*t37.*(t100-t364))+t2124.*(t100-t364)))+t3d.*(t4257+t4274-t5096+t14.*(t1862+t2375+t330.*(-t496-t547+t615+t623+t755+t8.*t37.*(t100-t364))+t2124.*(t100-t364)))+t4d.*(t4257+t4274-t5096+t14.*(t1862+t2375+t330.*(-t496-t547+t615+t623+t755+t8.*t37.*(t100-t364))+t2124.*(t100-t364))));
et89 = -t4d.*(-t4062-t5564+t5600+t2d.*(t4257+t4274-t5096+t14.*(t1862+t2375+t330.*(-t496-t547+t615+t623+t755+t8.*t37.*(t100-t364))+t2124.*(t100-t364)))+t3d.*(t4257+t4274-t5096+t14.*(t1862+t2375+t330.*(-t496-t547+t615+t623+t755+t8.*t37.*(t100-t364))+t2124.*(t100-t364)))+t4d.*(t4257+t4274-t5096+t14.*(t1862+t2375+t330.*(-t496-t547+t615+t623+t755+t8.*t37.*(t100-t364))+t2124.*(t100-t364))))+t3499.*t1dd-t4894.*t2dd-t4894.*t3dd-t4894.*t4dd-t5d.*(et83+et84)-t5dd.*(t3548+t3885+t3889)-t6dd.*(t3594+t3989+t4016);
et90 = t1d.*(-t1d.*(t187+t589)+t6d.*(t3532+(t256.*t1699)./2.0+(t329.*t1663)./2.0+(t255.*t2171)./2.0+(t330.*t2170)./2.0+t18.*t155.*t341+(t18.*t39.*t930)./2.0)+t5315.*t2d+t5315.*t3d+t5315.*t4d+t5d.*(t4526+(t37.*t930)./2.0+(t8.*t39.*t2170)./2.0-(t14.*t39.*t2171)./2.0))-t6d.*(et85+et86);
et91 = t1d.*(t1316./2.0-t2210./2.0+t2679./2.0+t3477./2.0)-t6d.*(t3594+t3989+t4016-(t329.*(t2782-t1070.*(t101-t401)))./2.0+t12.*t3711-(t256.*t3832)./2.0+(t255.*t5050)./2.0+(t330.*t5046)./2.0+(t18.*t39.*t4981)./2.0)+t2d.*(t3643+t3880-t3917-t5073-t5086+t5175-t5176+t18.*t39.*(-t1800+t2379+t2497+t18.*t39.*(-t495-t548+t650+t659+t739+t14.*t37.*(t101-t401))))+t3d.*(t3643+t3880-t3917-t5073-t5086+t5175-t5176+t18.*t39.*(-t1800+t2379+t2497+t18.*t39.*(-t495-t548+t650+t659+t739+t14.*t37.*(t101-t401))));
et92 = t4d.*(t3643+t3880-t3917-t5073-t5086+t5175-t5176+t18.*t39.*(-t1800+t2379+t2497+t18.*t39.*(-t495-t548+t650+t659+t739+t14.*t37.*(t101-t401))))+t5d.*(-t329.*(t2523-t1420.*(t101-t401))+t12.*t3611-t256.*t3789+t255.*t4727-(t37.*t4981)./2.0+t330.*t4722+t18.*t39.*t4528-(t8.*t39.*t5046)./2.0+(t14.*t39.*t5050)./2.0);
et93 = t1d.*(t191+t588)-t6d.*(t3499-(t256.*t1659)./2.0-(t329.*t1701)./2.0+(t330.*t2204)./2.0-(t255.*(-t537+t759+t12.*t39.*(t101-t401)))./2.0+t18.*t112.*t402+(t18.*t39.*t949)./2.0)+t2d.*(-t1800-t2327+t2379+t2497+(t8.*(-t537+t759+t12.*t39.*(t101-t401)))./2.0+t18.*t39.*(-t495-t548+t650+t659+t739+t14.*t37.*(t101-t401)))+t3d.*(-t1800-t2327+t2379+t2497+(t8.*(-t537+t759+t12.*t39.*(t101-t401)))./2.0+t18.*t39.*(-t495-t548+t650+t659+t739+t14.*t37.*(t101-t401)));
et94 = t4d.*(-t1800-t2327+t2379+t2497+(t8.*(-t537+t759+t12.*t39.*(t101-t401)))./2.0+t18.*t39.*(-t495-t548+t650+t659+t739+t14.*t37.*(t101-t401)))-t5d.*(-t4528+(t37.*t949)./2.0+(t8.*t39.*t2204)./2.0+(t14.*t39.*(-t537+t759+t12.*t39.*(t101-t401)))./2.0);
et95 = t6dd.*((t873-t2434).^2+(t910-t2473).^2+t2270.^2)+t4d.*(-t5d.*(-t4582+t5076+t2270.*(t745-t747)+t8.*t1807.*(t870-t909-t1470+t2472)+t8.*t1082.*(t873-t2434)+t14.*t1082.*(t910-t2473))+t4d.*(t3943-t4678-t4705+t4977+t8.*t1818.*(t873-t2434)+t14.*t1818.*(t910-t2473))+t3d.*(t4475-t4678-t4705+t4977+t8.*t1818.*(t873-t2434)+t14.*t1818.*(t910-t2473))+t2d.*(t4648-t4678-t4705+t4977+t8.*t1818.*(t873-t2434)+t14.*t1818.*(t910-t2473)));
et96 = t3d.*(-t5d.*(-t4668+t4935+t2270.*(t745-t747)+t8.*t2113.*(t870-t909-t1470+t2472)+t8.*t1082.*(t873-t2434)+t14.*t1082.*(t910-t2473))+t4d.*(t3943-t4747-t4759+t4815+t8.*t1818.*(t873-t2434)+t14.*t1818.*(t910-t2473))+t2d.*(t4348-t4747-t4759+t4815+t8.*t2140.*(t873-t2434)+t14.*t2140.*(t910-t2473))+t3d.*(t4348-t4747-t4759+t4815+t8.*t2140.*(t873-t2434)+t14.*t2140.*(t910-t2473)))-t1dd.*(t2658.*(t873-t2434)+t2654.*(t910-t2473));
et97 = -t2d.*(t5d.*(-t4707-t4971+t2270.*(t745-t747)+t8.*t2279.*(t870-t909-t1470+t2472)+t8.*t1082.*(t873-t2434)+t14.*t1082.*(t910-t2473))+t2d.*(t4776+t4798+t4879-t2270.*t3686+t8.*t2357.*(t873-t2434)+t14.*t2357.*(t910-t2473))+t3d.*(t4133+t4147+t4361+t4776+t4798+t4879)-t4d.*(t3943-t4776-t4798-t4879+t8.*t1818.*(t873-t2434)+t14.*t1818.*(t910-t2473)))-t5787.*t1d-t2dd.*(t4674+t8.*t2279.*(t873-t2434)+t14.*t2279.*(t910-t2473));
et98 = -t5d.*(-t5d.*(t1874.*t2270+t3081.*t3734-t3251.*t4178-t2169.*(t873-t2434)-t2123.*(t910-t2473)+t3230.*(t870-t909-t1470+t2472))+t2d.*(t4461+t4771+t4951+t4958+t4985+t4993)+t3d.*(t4461+t4771+t4951+t4958+t4985+t4993)+t4d.*(t4461+t4771+t4951+t4958+t4985+t4993))-t4dd.*(-t4868+t8.*t1807.*(t873-t2434)+t14.*t1807.*(t910-t2473))-t3dd.*(-t4561+t8.*t2113.*(t873-t2434)+t14.*t2113.*(t910-t2473));
et99 = t6d.*(t2d.*(t4171+t4335.*(t873-t2434).*2.0+t4353.*(t910-t2473).*2.0)+t3d.*(t4171+t4335.*(t873-t2434).*2.0+t4353.*(t910-t2473).*2.0)+t4d.*(t4171+t4335.*(t873-t2434).*2.0+t4353.*(t910-t2473).*2.0)-t5d.*(t2270.*t3734.*2.0+t4178.*(t910-t2473).*2.0-(t873-t2434).*(t870-t909-t1470+t2472).*2.0))+t5dd.*(-t4156+t3230.*(t873-t2434)+t3251.*(t910-t2473));
et100 = t4100+t5602-t5d.*(t4110+t4250+t4286+t37.*t4506+t8.*t39.*(t3377.*(t100-t364)+t13.*t330.*(t544-t1021+t330.*(t100-t364)))+t14.*t39.*t4575)+t2d.*(t2936+t3099-t4209+t4239+t4735+t755.*(t544-t1021+t330.*(t100-t364))+t14.*t39.*(t4074+t459.*(t544-t1021+t330.*(t100-t364)))+t8.*t39.*(t3804.*(t100-t364)+t453.*(t544-t1021+t330.*(t100-t364))))+t3d.*(t2936+t3099-t4209+t4239+t4735+t755.*(t544-t1021+t330.*(t100-t364))+t14.*t39.*(t4074+t459.*(t544-t1021+t330.*(t100-t364)))+t8.*t39.*(t3804.*(t100-t364)+t453.*(t544-t1021+t330.*(t100-t364))));
et101 = t4d.*(t2936+t3099-t4209+t4239+t4735+t755.*(t544-t1021+t330.*(t100-t364))+t14.*t39.*(t4074+t459.*(t544-t1021+t330.*(t100-t364)))+t8.*t39.*(t3804.*(t100-t364)+t453.*(t544-t1021+t330.*(t100-t364))));
et102 = t5d.*(et100+et101)+t5dd.*(t494.*(t544-t1021+t330.*(t100-t364))+t764.*(t544-t1021+t330.*(t100-t364))+t802.*(t544-t1021+t330.*(t100-t364)))-t2dd.*(t694.*(t544-t1021+t330.*(t100-t364))+t695.*(t544-t1021+t330.*(t100-t364)))-t3dd.*(t694.*(t544-t1021+t330.*(t100-t364))+t695.*(t544-t1021+t330.*(t100-t364)))-t4dd.*(t694.*(t544-t1021+t330.*(t100-t364))+t695.*(t544-t1021+t330.*(t100-t364)));
et103 = t1d.*(-t831+t5213+t5d.*(t943+t2387+t2479+t4506)+t2d.*(t2304+t2368-t4017+t403.*(t544-t1021+t330.*(t100-t364)))+t3d.*(t2304+t2368-t4017+t403.*(t544-t1021+t330.*(t100-t364)))+t4d.*(t2304+t2368-t4017+t403.*(t544-t1021+t330.*(t100-t364))))+t5792.*t2d+t5792.*t3d+t5792.*t4d;
et104 = t6d.*(t4370+t5428+t5675.*t2d+t5675.*t3d+t5675.*t4d-t5d.*(t4377+t4431+t4456+t330.*(t3377.*(t100-t364)+t13.*t330.*(t544-t1021+t330.*(t100-t364)))-t255.*t4575+t589.*(t544-t1021+t330.*(t100-t364))+t1066.*(t544-t1021+t330.*(t100-t364))+t1138.*(t544-t1021+t330.*(t100-t364))+t18.*t39.*t4506))+t6dd.*(t544.*(t544-t1021+t330.*(t100-t364))-t1021.*(t544-t1021+t330.*(t100-t364))+t330.*(t100-t364).*(t544-t1021+t330.*(t100-t364)))-t341.*t1dd.*(t544-t1021+t330.*(t100-t364));
et105 = t5dd.*(t546.*t2578+t726.*t2578+t871.*t2578)+t6dd.*(t591.*t2578+t1015.*t2578+t1069.*t2578)+t5d.*(t4114+t5605+t5662.*t2d+t5662.*t3d+t5662.*t4d+t5d.*(t4110+t4250+t4286+t37.*t4508+t8.*t39.*t4578-t14.*t39.*t4587))+t4408.*t2dd+t4408.*t3dd+t4408.*t4dd-t5793.*t2d-t5793.*t3d-t5793.*t4d-t1d.*(-t831+t5213+t5d.*(t943+t2387+t2479+t4508)+t5222.*t2d+t5222.*t3d+t5222.*t4d);
et106 = t6d.*(-t4370+t5427+t2d.*(t2991+t3098-t4419+t4762+t4850-t4857+t937.*t2578+(t14.*(t2578.*(t100-t364)+t609.*(t544-t1021+t330.*(t100-t364))))./2.0)+t3d.*(t2991+t3098-t4419+t4762+t4850-t4857+t937.*t2578+(t14.*(t2578.*(t100-t364)+t609.*(t544-t1021+t330.*(t100-t364))))./2.0)+t4d.*(t2991+t3098-t4419+t4762+t4850-t4857+t937.*t2578+(t14.*(t2578.*(t100-t364)+t609.*(t544-t1021+t330.*(t100-t364))))./2.0)+t5d.*(t4377+t4431+t4456+t588.*t2578+t1017.*t2578+t1193.*t2578+t255.*t4587+t330.*t4578+t18.*t39.*t4508))-t402.*t2578.*t1dd;
et107 = -t5d.*(-t5d.*((t37.*t4078)./2.0-t37.*t5257+t14.*t39.*(t2816+t3757+t3780-t19.*t255.*(t544-t1021+t330.*(t100-t364)))-t8.*t39.*(t2853+t3739+t3755-t19.*t330.*(t544-t1021+t330.*(t100-t364)))-(t8.*t39.*t4168)./2.0+(t14.*t39.*t4196)./2.0)-t6d.*(t37.*t4331-(t255.*t4196)./2.0-(t330.*t4168)./2.0+(t18.*t39.*t4078)./2.0+t8.*t39.*t4402+t14.*t39.*t4410)+t5765.*t2d+t5765.*t3d+t5765.*t4d+t1d.*(t341.*t2198-t402.*t2233))-t2d.*(-t3327+t5499+t5631+t2d.*(t3652-t3691-t5369+t5373)+t3d.*(t3652-t3691-t5369+t5373)+t4d.*(t3652-t3691-t5369+t5373));
et108 = -t3d.*(-t3327+t5499+t5631+t2d.*(t3652-t3691-t5369+t5373)+t3d.*(t3652-t3691-t5369+t5373)+t4d.*(t3652-t3691-t5369+t5373))-t4d.*(-t3327+t5499+t5631+t2d.*(t3652-t3691-t5369+t5373)+t3d.*(t3652-t3691-t5369+t5373)+t4d.*(t3652-t3691-t5369+t5373))-t4330.*t1dd-t5243.*t2dd-t5243.*t3dd-t5243.*t4dd+t6dd.*(t18.*t4364-t255.*t4404+t330.*(t2578.*(t100-t364)+t609.*(t544-t1021+t330.*(t100-t364))))+t5dd.*(t4363+t4421+t4433);
et109 = t6d.*(t5768.*t2d+t5768.*t3d+t5768.*t4d+t1d.*(t402.*t2578-t341.*(t544-t1021+t330.*(t100-t364)))+t6d.*(t255.*t4410.*(-1.0./2.0)+(t330.*t4402)./2.0+(t18.*t39.*t4331)./2.0)-t5d.*((t37.*t4331)./2.0-t12.*t4364-t329.*t4404+t256.*(t2578.*(t100-t364)+t609.*(t544-t1021+t330.*(t100-t364)))+t255.*(t2816+t3757+t3780-t19.*t255.*(t544-t1021+t330.*(t100-t364)))+t330.*(t2853+t3739+t3755-t19.*t330.*(t544-t1021+t330.*(t100-t364)))+(t8.*t39.*t4402)./2.0+(t14.*t39.*t4410)./2.0+t18.*t39.*t5257));
et110 = t1d.*(t2d.*(t2305+t2369+t2878-t4023-t4038+t342.*(t544-t1021+t330.*(t100-t364)))+t3d.*(t2305+t2369+t2878-t4023-t4038+t342.*(t544-t1021+t330.*(t100-t364)))+t4d.*(t2305+t2369+t2878-t4023-t4038+t342.*(t544-t1021+t330.*(t100-t364)))+t6d.*(-t2895+(t255.*t2259)./2.0+(t330.*t2190)./2.0+t341.*(t544-t1021+t330.*(t100-t364)).*2.0-(t18.*t39.*t1044)./2.0)-t5d.*(-t2699+t3607-t3624+(t37.*t1044)./2.0+t18.*t63.*(t544-t1021+t330.*(t100-t364))-(t8.*t39.*t2190)./2.0+(t14.*t39.*t2259)./2.0)+t1d.*(t418-t446));
et111 = -t5d.*(t3609./2.0+t3861./2.0-t3888./2.0+t37.*t4975+t8.*t39.*t5049-t14.*t39.*t5045)-t6d.*(t3647./2.0-t3669-t3944+t3962+t4005./2.0+t4007./2.0)+t2d.*(-t3670-t3839-t3858+t3927+t5145+t37.*(-t1537+t1983+t3892+t18.*t37.*(t544-t1021+t330.*(t100-t364)))+t8.*t37.*(t1070.*(t100-t364)+t330.*(t544-t1021+t330.*(t100-t364)))+t14.*t39.*(t1585+t2193-t4001+t38.*t39.*(t544-t1021+t330.*(t100-t364))));
et112 = t3d.*(-t3670-t3839-t3858+t3927+t5145+t37.*(-t1537+t1983+t3892+t18.*t37.*(t544-t1021+t330.*(t100-t364)))+t8.*t37.*(t1070.*(t100-t364)+t330.*(t544-t1021+t330.*(t100-t364)))+t14.*t39.*(t1585+t2193-t4001+t38.*t39.*(t544-t1021+t330.*(t100-t364))))+t4d.*(-t3670-t3839-t3858+t3927+t5145+t37.*(-t1537+t1983+t3892+t18.*t37.*(t544-t1021+t330.*(t100-t364)))+t8.*t37.*(t1070.*(t100-t364)+t330.*(t544-t1021+t330.*(t100-t364)))+t14.*t39.*(t1585+t2193-t4001+t38.*t39.*(t544-t1021+t330.*(t100-t364))));
et113 = t1d.*(t1829./2.0+t2382./2.0);
et114 = -t5dd.*(t3668+t3931+t8.*t39.*(t1070.*(t100-t364)+t330.*(t544-t1021+t330.*(t100-t364))))+t3602.*t1dd+t4915.*t2dd+t4915.*t3dd+t4915.*t4dd+t5799.*t2d+t5799.*t3d+t5799.*t4d-t6dd.*(t18.*t3670-t255.*t3833+t330.*(t1070.*(t100-t364)+t330.*(t544-t1021+t330.*(t100-t364))))-t5d.*(et111+et112+et113)-t1d.*(-t591.*t1d+t5265.*t2d+t5265.*t3d+t5265.*t4d+t5d.*(t1816./2.0-t1835./2.0+t4975+t174.*t402)+t6d.*(t2059./2.0+t2061./2.0-t3603+t137.*t402));
et115 = -t6d.*(-t5d.*(t3669./2.0+t3944./2.0-t3962./2.0-t12.*t3670-t329.*t3833+t255.*t5045+t330.*t5049+t256.*(t1070.*(t100-t364)+t330.*(t544-t1021+t330.*(t100-t364)))+t18.*t39.*t4975)+t5695.*t2d+t5695.*t3d+t5695.*t4d+t1d.*(t1536./2.0+t2681./2.0)+t6d.*((t255.*(t2782-t1070.*(t101-t401)))./2.0+t18.*t3711+(t330.*t3832)./2.0));
et116 = -t6d.*(t5696.*t2d+t5696.*t3d+t5696.*t4d-t6d.*(t18.*t3710-(t255.*t3833)./2.0+(t330.*(t1070.*(t100-t364)+t330.*(t544-t1021+t330.*(t100-t364))))./2.0)-t1d.*(t1504./2.0+t2705./2.0)+t5d.*(t3668./2.0+t3931./2.0-t329.*(t2782-t1070.*(t101-t401))+t12.*t3671-t256.*t3832+t255.*t5050+t330.*t5046+(t8.*t39.*(t1070.*(t100-t364)+t330.*(t544-t1021+t330.*(t100-t364))))./2.0+t18.*t39.*t4981))+t3603.*t1dd-t4916.*t2dd-t4916.*t3dd-t4916.*t4dd+t5800.*t2d+t5800.*t3d+t5800.*t4d;
et117 = t1d.*(t593.*t1d+t5268.*t2d+t5268.*t3d+t5268.*t4d+t6d.*(-t1504+t2022./2.0+t2086./2.0+t2682+t137.*t341)+t5d.*(t1803.*(-1.0./2.0)+t1848./2.0+t4981+t174.*t341))-t5d.*(t5691.*t2d+t5691.*t3d+t5691.*t4d-t6d.*(t3594.*(-1.0./2.0)+t3668+t3931-t4016./2.0+(t255.*(t2068-t2488))./2.0+t8.*t39.*(t1070.*(t100-t364)+t330.*(t544-t1021+t330.*(t100-t364))))+t5d.*(t3548./2.0+t3885./2.0+t3889./2.0+t37.*t4981+t8.*t39.*t5046-t14.*t39.*t5050)-t1d.*(t1799./2.0+t2358./2.0))-t6dd.*(t255.*(t2782-t1070.*(t101-t401))+t18.*t3671+t330.*t3832);
et118 = -t5dd.*(t3669+t3944-t3962);
mt1 = [t1dd.*(t23.*4.0513225e-3+t26.*4.0513225e-3),0.0,0.0,0.0,0.0,0.0,-t1519.*t2dd-t22.*(t127.*t454+t124.*t486)+t1dd.*(t454.^2+t486.^2)-t1d.*t2d.*(t15.*t532.*(1.53e+2./1.25e+2)-t15.*t554.*(1.53e+2./1.25e+2))];
mt2 = [t244+t2d.*(t1534.*t1d+t2d.*(t15.*t48.*3.74544e-1+t15.*t50.*3.74544e-1-t1203.*(t51.*(1.53e+2./2.5e+2)+t55.*(1.53e+2./2.5e+2))))-t1d.*(t1534.*t2d-t1d.*(t15.*t532.*(1.53e+2./2.5e+2)-t134.*t486))-t1519.*t1dd+t2dd.*(t23.*t27.*3.74544e-1+t26.*t27.*3.74544e-1+t1203.^2),0.0,0.0,0.0,0.0];
mt3 = [-t2374.*t3dd-t2719.*t2dd-t2d.*(t2405+t2d.*(t14.*t529.*t793+t8.*t529.*t824))-t1d.*(t2d.*((t299.*t884)./5.0e+3-(t299.*t928)./5.0e+3)+t3d.*(t31.*t884.*1.1446-t31.*t928.*1.1446))+t1dd.*(t793.^2+t824.^2)-t3d.*(t2405+t2371.*t2d),et17+et18,et31+et32,0.0,0.0,0.0];
mt4 = [-t3d.*(t3460+t2d.*(t2075+t2119+t2353+t2354)+t3d.*(t2353+t2354-t14.*t647.*t1121+t8.*t647.*t1140))+t3429.*t4dd+t3817.*t3dd+t4025.*t2dd-t4d.*(t3460+t3d.*(t1500+t1516+t3431)+t2d.*(t1740+t1759+t3431))-t2d.*(t3460+t3d.*(t2044+t2074+t2353+t2354)-t2d.*(-t8.*t820.*t1413+t14.*t820.*t1410+t8.*t843.*t1677+t14.*t843.*t1674))+t1dd.*(t1674.^2+t1677.^2)+t1d.*(t4d.*(t37.*t1736.*1.639e-1-t37.*t171.*t1677)+t3d.*(t1121.*t1674.*2.0-t1140.*t1677.*2.0)+t2d.*(t1410.*t1674.*2.0-t1413.*t1677.*2.0)),et19+et20,et33+et34,et44+et45,0.0,0.0,et1+et2,et21+et22+et23+et24,et35+et36+et37,et46+et47+et48,et55+et56+et57,0.0,et3+et4,et25+et26+et27+et28+et29+et30,et38+et39+et40+et41+et42+et43];
mt5 = [et49+et50+et51+et52+et53+et54,et60+et61+et62+et63+et64,et95+et96+et97+et98+et99,0.0,0.0,0.0,0.0,0.0,0.0,t1dd,0.0,0.0,0.0,0.0,0.0,0.0,0.0,0.0,0.0,0.0,0.0,0.0,0.0,0.0,0.0,0.0,0.0,0.0,0.0,0.0,0.0,0.0,0.0,0.0,0.0,0.0,0.0,0.0,0.0,t58+t972+t27.*t1dd,-t1266,0.0,0.0,0.0,0.0,-t58-t972+t24.*t1dd,t1266,0.0,0.0,0.0,0.0,0.0,t617,0.0,0.0,0.0,0.0,t853.*t2dd+t1d.*t2d.*(t24.*2.0-t27.*2.0)+t9.*t15.*t1dd.*2.0,-t21.*(t24-t27),0.0,0.0,0.0,0.0,t22.*t226+t229.*t2dd,-t1d.*t2d.*(t48./2.0+t50./2.0-t9.*t82)+t15.*t82.*t1dd-(t9.*t82.*t1d.*t2d)./2.0,0.0,0.0,0.0,0.0,-t22.*t229+t226.*t2dd];
mt6 = [t1d.*t2d.*(t51./2.0+t55./2.0-t15.*t82)+t9.*t82.*t1dd+(t15.*t82.*t1d.*t2d)./2.0,0.0,0.0,0.0,0.0,t497+t2223+t2224+t42.*t1dd,t2603,t2603,0.0,0.0,0.0,-t497-t2223-t2224+t41.*t1dd,t2570,t2570,0.0,0.0,0.0,0.0,t1368,t1368,0.0,0.0,0.0,t1071.*t2dd+t1071.*t3dd+t1d.*(t318.*t2d+t318.*t3d)+t30.*t31.*t1dd.*2.0,t434,t434,0.0,0.0,0.0,t343.*t2dd+t343.*t3dd+t865.*t2d+t865.*t3d,t2795,t2795,0.0,0.0,0.0,t365.*t2dd+t365.*t3dd-t842.*t2d-t842.*t3d,t2731,t2731,0.0,0.0,0.0,t828+t3170+t3171+t3172+t56.*t1dd,t3505,t3505,t3505,0.0,0.0,0.0,t1984,t1984,t1984,0.0,0.0,t75+t879+t3209+t3210+t3211,t3486,t3486,t3486,0.0,0.0,t431.*t2dd+t431.*t3dd+t431.*t4dd+t1485.*t2d+t1485.*t3d+t1485.*t4d,t3732,t3732,t3732,0.0,0.0,0.0,0.0,0.0,0.0,0.0];
mt7 = [0.0,-t425.*t2dd-t425.*t3dd-t425.*t4dd+t1492.*t2d+t1492.*t3d+t1492.*t4d,t3754,t3754,t3754,0.0,0.0,t1186.*t2dd+t1186.*t3dd+t1186.*t4dd+t4653.*t2d+t4653.*t3d+t4653.*t4d+t1d.*(t25.*t163+t25.*t164+t25.*t165+t200.*t5d)-t5d.*(t2d.*(-t132+t319-t614+t655+t1026+t8.*t39.*(t206-t470))+t3d.*(-t132+t319-t614+t655+t1026+t8.*t39.*(t206-t470))+t4d.*(-t132+t319-t614+t655+t1026+t8.*t39.*(t206-t470))+t5d.*(t1317+t37.*t200+t8.*t39.*(t478-t519)))-t5dd.*(t199.*t256+t150.*t329+t25.*t37.*t56)+t25.*t56.*t1dd,t5797,t5797,t5797];
mt8 = [t5dd.*(t173.*t1419+t516.*t1419+t523.*t1419)-t3151.*t2dd-t3151.*t3dd-t3151.*t4dd-t5688.*t2d-t5688.*t3d-t5688.*t4d+t5d.*(t2990+t5017+t2d.*(-t1615+t1919+t1921+t3218+t3220+t3376+t3533+t3559)+t3d.*(-t1615+t1919+t1921+t3218+t3220+t3376+t3533+t3559)+t4d.*(-t1615+t1919+t1921+t3218+t3220+t3376+t3533+t3559))-t1d.*(t220+t4297+t4317.*t2d+t4317.*t3d+t4317.*t4d)+t12.*t1569.*t1dd,0.0,t75+t879+t3209+t3210+t3211-t5d.*(t2281.*t2d+t2281.*t3d+t2281.*t4d)-t5dd.*(t56.*t104+t56.*t107+t37.^3),t5541,t5541,t5541];
mt9 = [t5dd.*(t53.*t637+t131.*t637+t136.*t637)+t5d.*(t4858.*t2d+t4858.*t3d+t4858.*t4d)+t5202.*t2d+t5202.*t3d+t5202.*t4d+t1d.*(t2d.*(t738-t1085)+t3d.*(t738-t1085)+t4d.*(t738-t1085))-t37.*t637.*t1dd,0.0,t175+t1271+t1272+t1273+t1461+t1715+t4696+t4697+t4698+t5285,t5798,t5798,t5798];
mt10 = [t1617+t3195+t3196+t3197+t4087+t5689.*t2d+t5689.*t3d+t5689.*t4d+t5d.*(t2962+t5016+t2d.*(-t1586-t1867+t1920-t3218+t3370+t3535+(t14.*(t1743-t1783))./2.0+t14.*t39.*(t1609-t2416))+t3d.*(-t1586-t1867+t1920-t3218+t3370+t3535+(t14.*(t1743-t1783))./2.0+t14.*t39.*(t1609-t2416))+t4d.*(-t1586-t1867+t1920-t3218+t3370+t3535+(t14.*(t1743-t1783))./2.0+t14.*t39.*(t1609-t2416)))-t1d.*(t162+t4272+t2d.*(-t1281+t3322+(t14.*(t478-t519))./2.0)+t3d.*(-t1281+t3322+(t14.*(t478-t519))./2.0)+t4d.*(-t1281+t3322+(t14.*(t478-t519))./2.0)),0.0];
mt11 = [t1687.*t2dd+t1687.*t3dd+t1687.*t4dd-t2222.*t5dd-t4509.*t2d-t4509.*t3d-t4509.*t4d+t1d.*(t174.*t5d.*-2.0+t487.*t2d+t487.*t3d+t487.*t4d)-t5d.*(-t2225.*t5d+t2d.*(t601+t922+t959+t963+t1087+t37.*t156)+t3d.*(t601+t922+t959+t963+t1087+t37.*t156)+t4d.*(t601+t922+t959+t963+t1087+t37.*t156))+t12.*t152.*t1dd,t5788,t5788,t5788];
mt12 = [-t1d.*(-t18.*t128+t4532.*t2d+t4532.*t3d+t4532.*t4d+t5d.*(t923./2.0+t973./2.0-t2308+t39.*t111))-t2306.*t1dd-t4061.*t2dd-t4061.*t3dd-t4061.*t4dd+t5647.*t2d+t5647.*t3d+t5647.*t4d+t5d.*(t5542.*t2d+t5542.*t3d+t5542.*t4d-t1d.*(t776./2.0+t1528./2.0)-t5d.*((t37.*t2308)./2.0+(t8.*t39.*t2513)./2.0-(t14.*t39.*t2514)./2.0))+t5dd.*(t37.*t2306-t8.*t39.*t2510+t14.*t39.*t2512),0.0];
mt13 = [t200.*t1dd+t2296.*t2dd+t2296.*t3dd+t2296.*t4dd-t5058.*t2d-t5058.*t3d-t5058.*t4d-t1d.*(t570.*t5d+t18.*t173.*t2d.*4.0+t18.*t173.*t3d.*4.0+t18.*t173.*t4d.*4.0)-t5d.*(t2d.*(t177-t333+t1312-t1599-t1607+t8.*t37.*(t478-t519))+t3d.*(t177-t333+t1312-t1599-t1607+t8.*t37.*(t478-t519))+t4d.*(t177-t333+t1312-t1599-t1607+t8.*t37.*(t478-t519))-t5d.*(t37.*t570-t8.*t39.*t1128+t14.*t39.*t1129))-t5dd.*(t1317+t37.*t200+t8.*t39.*(t478-t519)),t5831,t5831,t5831];
mt14 = [t5dd.*(-t37.*t2828+t14.*t39.*t3104+t8.*t39.*(t1743-t1783))+t1d.*(-t5d.*(-t1578+t1579+(t37.*t570)./2.0-(t8.*t39.*t1128)./2.0+(t14.*t39.*t1129)./2.0)+t4953.*t2d+t4953.*t3d+t4953.*t4d-t1d.*(t137-t25.*t56))+t2828.*t1dd-t4492.*t2dd-t4492.*t3dd-t4492.*t4dd-t5754.*t2d-t5754.*t3d-t5754.*t4d-t5d.*(t5d.*((t37.*(t1578-t1579))./2.0-(t8.*t39.*t3106)./2.0+(t14.*t39.*t3107)./2.0)+t5610.*t2d+t5610.*t3d+t5610.*t4d+t1d.*(t12.*t1529+t18.*t1571)),0.0];
mt15 = [t174.*t1dd.*-2.0+t1692.*t2dd+t1692.*t3dd+t1692.*t4dd+t2225.*t5dd-t4503.*t2d-t4503.*t3d-t4503.*t4d+t5d.*(t2222.*t5d+t2d.*(t608+t919+t965+t970+t1086+t37.*t159)+t3d.*(t608+t919+t965+t970+t1086+t37.*t159)+t4d.*(t608+t919+t965+t970+t1086+t37.*t159))-t1d.*(t488.*t2d+t488.*t3d+t488.*t4d+t12.*t152.*t5d),t5789,t5789,t5789];
mt16 = [t1d.*(t12.*t128+t4537.*t2d+t4537.*t3d+t4537.*t4d-t5d.*(t927./2.0+t966./2.0-t2306+t39.*t106))+t2308.*t1dd-t4063.*t2dd-t4063.*t3dd-t4063.*t4dd-t5d.*(t5543.*t2d+t5543.*t3d+t5543.*t4d+t1d.*(t775./2.0+t1525./2.0)+t5d.*((t37.*t2306)./2.0-(t8.*t39.*t2510)./2.0+(t14.*t39.*t2512)./2.0))-t2d.*(-t1049+t4821+t5191+t5192+t5193)-t3d.*(-t1049+t4821+t5191+t5192+t5193)-t4d.*(-t1049+t4821+t5191+t5192+t5193)-t5dd.*(t37.*t2308+t8.*t39.*t2513-t14.*t39.*t2514),0.0,et5+et6,t5838,t5838,t5838,et70+et71,et102+et103+et104,et7+et8,t5839,t5839,t5839,et72+et73+et74+et75,et105+et106];
mt17 = [t175+t1271+t1272+t1273+t1461+t1715+t4696+t4697+t4698+t5285-t6d.*(-t5d.*(t12.*t138.*-3.0+t330.*t478-t255.*t1126+t330.*(t478-t519)+t18.*t329.*t437)+t3502.*t2d+t3502.*t3d+t3502.*t4d)-t6dd.*(t29.*t57+t18.*t39.*t317+t18.*t39.*t368),t5822,t5822,t5822,et76+et77+et78];
mt18 = [t6d.*(t5267.*t2d+t5267.*t3d+t5267.*t4d-t5d.*(t255.*t1497+t330.*t1468+t255.*t3175+t330.*t3176+t18.*t155.*t1070-t18.*t39.*(t1268-t1988)))+t6dd.*(t137.*t1070+t317.*t1070+t368.*t1070)+t5dd.*(t174.*t1070+t514.*t1070+t524.*t1070)+t5d.*(t5d.*(t37.*(t1268-t1988)-t8.*t39.*t3176+t14.*t39.*t3175)+t5256.*t2d+t5256.*t3d+t5256.*t4d)+t2737.*t2dd+t2737.*t3dd+t2737.*t4dd+t5494.*t2d+t5494.*t3d+t5494.*t4d-t1d.*(t2722.*t2d+t2722.*t3d+t2722.*t4d+t5d.*(t1268-t1988))-t18.*t39.*t1070.*t1dd,et9+et10+et11+et12,t5842,t5842,t5842,et81+et82,et107+et108+et109+et110,et13+et14,t5840,t5840,t5840,et87+et88+et89+et90,et114+et115,et15+et16,t5841,t5841,t5841];
mt19 = [t5d.*(t5711.*t2d+t5711.*t3d+t5711.*t4d-t1d.*(t1610./2.0+t1680./2.0+t1827./2.0+t2380./2.0)+t6d.*(t3548+t3885+t3889-(t329.*(t2523-t1420.*(t101-t401)))./2.0+t12.*t3648-(t256.*t3789)./2.0+(t255.*t4727)./2.0+(t330.*t4722)./2.0+(t18.*t39.*t4528)./2.0)-t5d.*((t37.*t4528)./2.0+(t8.*t39.*t4722)./2.0-(t14.*t39.*t4727)./2.0))+t3532.*t1dd-t4895.*t2dd-t4895.*t3dd-t4895.*t4dd+t5809.*t2d+t5809.*t3d+t5809.*t4d-t5dd.*(t3609+t3861+t3919)-t6dd.*(t3647+t4005+t4007)-t6d.*(et91+et92)+t1d.*(et93+et94),et116+et117+et118];
Y = reshape([mt1,mt2,mt3,mt4,mt5,mt6,mt7,mt8,mt9,mt10,mt11,mt12,mt13,mt14,mt15,mt16,mt17,mt18,mt19],6,42);
end
